simulink subsystem "simscape_thermofluids_full_subsystem"  (R2024b)
settings: Solver=VariableStepAuto  StartTime=0.0  StopTime=10.0  RelTol=1e-3
values from neighbouring files (symbols this model uses):
  Ambient_temp = 300    [design_details.m]
  hose_length = 20    [design_details.m]
  Initial_temp = 300    [design_details.m]
  mass_per_length_return = steel_density*wall_thickness*(return_pipe_inner_area + return_pipe_outer_area)    [design_details.m]
  mass_per_length_supply = steel_density*wall_thickness*(supply_pipe_inner_area + supply_pipe_outer_area)    [design_details.m]
  return_pipe_inner_diameter = 0.1    [design_details.m]
  supply_pipe_inner_diameter = 0.1    [design_details.m]
  wall_thickness = 2/1000    (= 0.002)    [design_details.m]
undefined symbols (not defined in the file or in its folder): AC_bypass_line_Mdot, AC_bypass_line_Qdot, AC_Bypass_SOV_POS, AC_Engine_SOV_POS, AC_return_coupling_Qdot, AC_return_line_Mdot, AC_return_line_Qdot, AC_Return_SOV_POS, AC_supply_coupling_Qdot, AC_supply_line_Mdot, AC_supply_line_Qdot, AC_Supply_SOV_POS, AC_Tank_return_line_mdot, AC_Tank_return_line_Qdot, AC_TANK_SUPPLY_LINE_MDOT, AC_TANK_SUPPLY_LINE_QDOT, AC_Tank_Vent_mdot, AC_Tank_Vent_Qdot, Engine_feed_mdot, Engine_feed_Qdot, GH2_PROP_VALVE_POS, GS_GH2_RETURN_PROP_POS, GS_GH2_RETURN_SOV_POS, GS_GH2_SOV_POS, GS_LH2_Return_SOV_POS, GS_RETURN_PROP_POS, GS_Supply_SOV_POS, LH2_PROP_VALVE_POS, P_BYPASS, P_COUPLING_AC, P_COUPLING_AC_RETURN, P_COUPLINGS_GS, P_ENGINE_FEED, P_GAS_RETURN, P_GH2_SUPPLY_GS, P_HOSE_GS, P_HOSE_RETURN_GS, P_PUMP_GS, P_TANK_AC, P_TANK_GS, P_VALVE_GS, P_VALVE_RETURN_GS, T_BYPASS, T_COUPLING_AC, T_COUPLING_AC_RETURN, T_COUPLINGS_GS, T_ENGINE_FEED, T_GAS_RETURN, T_GH2_SUPPLY_GS, T_HOSE_GS, T_HOSE_RETURN_GS, T_PUMP_GS, T_TANK_AC, T_TANK_GS, T_VALVE_GS, T_VALVE_RETURN_GS
libraries: nesl_utility x85, fl_lib x83, SimscapeFluids_lib x17
(part 1 of 2)
settings Model: Creator=MW  LastModifiedBy=MW

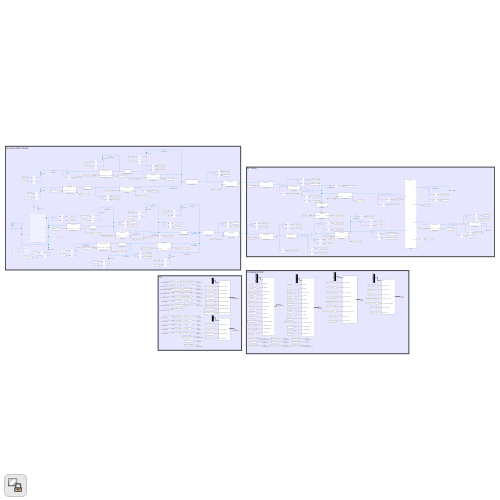
[thumbnail: Simulink's stored preview of the top-level diagram]
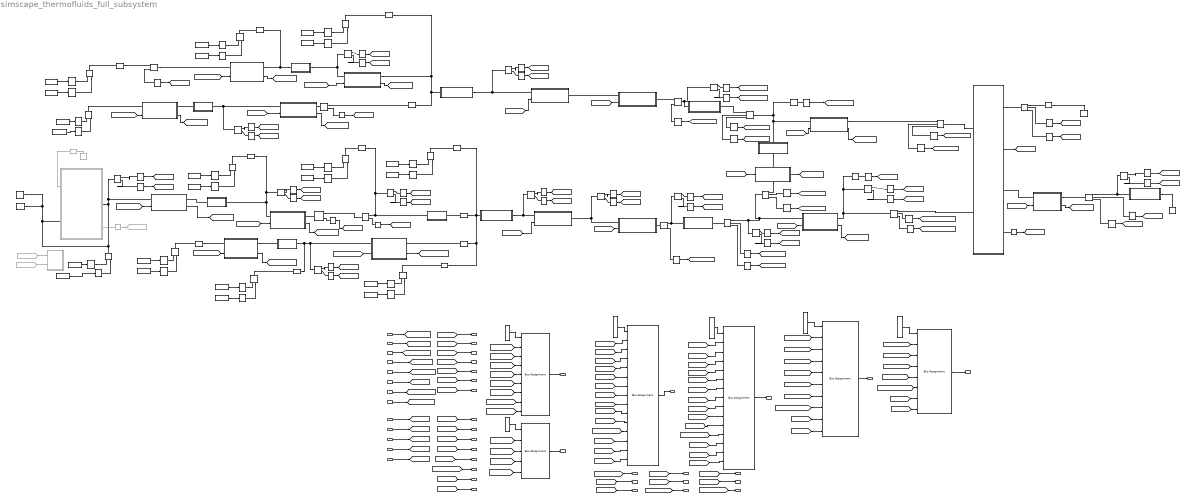
== system simscape_thermofluids_full_subsystem ==
  note: AC fluids
  note: Ground station fluids
  note: DIAGNOSTICS
  note: I/O
  LH2_PROP_VALVE_CMD : Inport  OutDataTypeStr=double
  GH2_PROP_VALVE_CMD : Inport  Port=2
  LH2 VENT PROP VALVE CMD : Inport  Port=3
  GS_LH2_Supply_SOV_CMD : Inport  Port=4  OutDataTypeStr=boolean
  GS_LH2_Return_SOV_CMD : Inport  Port=5  OutDataTypeStr=boolean
  GS_GH2_SOV_CMD : Inport  Port=6  OutDataTypeStr=boolean
  Couplings_connected : Inport  Port=7  OutDataTypeStr=boolean
  AC_Bypass_SOV_CMD : Inport  Port=8  OutDataTypeStr=boolean
  AC_Supply_SOV_CMD : Inport  Port=9  OutDataTypeStr=boolean
  AC_Return_SOV_CMD : Inport  Port=10  OutDataTypeStr=boolean
  AC_Engine_SOV_CMD : Inport  Port=11  OutDataTypeStr=boolean
  GS_GH2_RETURN_SOV_CMD : Inport  Port=12  OutDataTypeStr=boolean
  GH2_VENT_PROP_VALVE_CMD : Inport  Port=13
  AC bypass pipe : Subsystem  ReferencedSubsystem=AC_bypass_pipe
      settings: PortSchema="{\"entries\":[{\"content\":{\"sides\":[{\"content\":{},\"type\":\"ConnectorPlacement.EquallySpacedRectSide\",\"uuid\":\"f855fa5c-e5c1-49a4-a4bd-bb526208fa5d\"},{\"content\":{\"side\":\"RIGHT\"},\"type\":\"ConnectorPlacement.EquallySpacedRectSide\",\"uuid\":\"38379b5c-3270-47da-8350-930eb7311903\"},{\"content\":{\"connectorIds\":[\"RConn1\"],\"side\":\"TOP\"},\"type\":\"ConnectorPlacement.EquallySpacedRectSide\",\"uuid\":\"bb5b7562-7a02-4290-8016-95c457fb0f4b\"},{\"content\":{\"connectorIds\":[\"LConn1\"],\"side\":\"BOTTOM\"},\"type\":\"ConnectorPlacement.EquallySpacedRectSide\",\"uuid\":\"44fc2626-0acf-483b-8317-5c56b92a9255\"}]},\"type\":\"ConnectorPlacement.EquallySpacedConnector\",\"uuid\":\"6c85636f-b857-4cac-a183-27922e813604\"}],\"packageUris\":[\"http://schema.mathworks.com/mf0/Connector/R2020b\"],\"version\":\"1.0\"}"
  AC engine feed pipe : Subsystem  ReferencedSubsystem=AC_engine_line_pipe
  AC return line pipe : Subsystem  ReferencedSubsystem=AC_return_line_pipe
  AC return vapour quality : fl_lib/Two-Phase Fluid/Sensors/Vapor Quality Sensor (2P)  vapor_fraction_spec=foundation.enum.vapor_fraction_spec.quality
      settings: InternalSimscapePortConfiguration="{\"Bottom\":[],\"Left\":[{\"id\":\"A\",\"label\":\"A\",\"type\":\"foundation.two_phase_fluid.two_phase_fluid\"}],\"Right\":[{\"id\":\"X\",\"label\":\"X\",\"type\":\"output\"}],\"Top\":[]}"
  AC supply line quality : fl_lib/Two-Phase Fluid/Sensors/Vapor Quality Sensor (2P)  vapor_fraction_spec=foundation.enum.vapor_fraction_spec.quality
      settings: InternalSimscapePortConfiguration="{\"Bottom\":[],\"Left\":[{\"id\":\"A\",\"label\":\"A\",\"type\":\"foundation.two_phase_fluid.two_phase_fluid\"}],\"Right\":[{\"id\":\"X\",\"label\":\"X\",\"type\":\"output\"}],\"Top\":[]}"
  AC tank : Subsystem  ReferencedSubsystem=AC_tank
      settings: PortSchema="{\"entries\":[{\"content\":{\"sides\":[{\"content\":{\"connectorIds\":[\"LConn1\",\"LConn2\"]},\"type\":\"ConnectorPlacement.EquallySpacedRectSide\",\"uuid\":\"18fbfd65-7892-4f33-871e-6daf68ba144c\"},{\"content\":{\"connectorIds\":[\"RConn1\",\"Out1\",\"RConn2\",\"RConn3\"],\"side\":\"RIGHT\"},\"type\":\"ConnectorPlacement.EquallySpacedRectSide\",\"uuid\":\"09c519c2-126c-4ac0-b88b-b8c0f8bd496e\"},{\"content\":{\"side\":\"TOP\"},\"type\":\"ConnectorPlacement.EquallySpacedRectSide\",\"uuid\":\"0da44e65-d94a-4bbc-a863-04d0cc4fadcc\"}]},\"type\":\"ConnectorPlacement.EquallySpacedConnector\",\"uuid\":\"f3f4eab3-fa1f-4341-9602-c44ab5467c31\"}],\"packageUris\":[\"http://schema.mathworks.com/mf0/Connector/R2020b\"],\"version\":\"1.0\"}"
  AC tank safety valve : SimscapeFluids_lib/Two-Phase Fluid/Valves & Orifices/Directional Control Valves/Check Valve (2P)  liquid_valve_parameterization=fluids.two_phase_fluid.valves_orifices.enum.LiquidPressureValveParameterization.LinearArea  opening_pressure_spec=fluids.two_phase_fluid.valves_orifices.enum.PressureControlSpec.PressureDifferential  p_crack_differential=4.5 bar  p_crack_gauge=0.1 MPa  p_max_differential=4.9 bar  p_max_gauge=0.2 MPa  mdot_nominal_max=0.1 kg/s  delta_p_nominal_max=0.001 MPa  valve_area_max=AC_vent_valve_orifice_area m^2  p_diff_TLU=[0.2 : 0.2 : 1.2] MPa  p_gauge_TLU=[0.2 : 0.2 : 1.2] MPa  valve_area_TLU=[1e-10, 2e-06, 4e-06, 6e-06, 8e-06, 1e-05] m^2  energy_spec=foundation.enum.energy_spec.temperature  p_inlet=0.101325 MPa  T_inlet=293.15 K  x_inlet=0  alpha_inlet=0  h_inlet=400 kJ/kg  u_inlet=400 kJ/kg  Cd=AC_vent_valve_discharge_coeff  pressure_recovery=false  leakage_fraction=1e-9  smoothing_factor=0.01  B_lam=0.999  tau_x=0.1 s  area=AC_vent_line_port_inner_area m^2  vapor_valve_parameterization=fluids.two_phase_fluid.valves_orifices.enum.VaporOrificeParameterization.Cv  opening_characteristic=fluids.two_phase_fluid.valves_orifices.enum.OpeningCharacteristics.Linear  Cv_max=4  p_diff_Cv_TLU=0.2 : 0.2 : 1.2 MPa  p_gauge_Cv_TLU=0.2 : 0.2 : 1.2 MPa  Cv_TLU=[1e-06, .8, 1.6, 2.4, 3.2, 4]  xT_Cv=0.7  Kv_max=3.6  p_diff_Kv_TLU=0.2 : 0.2 : 1.2 MPa  p_gauge_Kv_TLU=0.2 : 0.2 : 1.2 MPa  Kv_TLU=[1e-06, .72, 1.44, 2.16, 2.88, 3.6]  xT_Kv=0.7  orifice_area_max=1e-4 m^2  p_diff_orifice_area_TLU=0.2 : 0.2 : 1.2 MPa  p_gauge_orifice_area_TLU=0.2 : 0.2 : 1.2 MPa  orifice_area_TLU=[1e-10, 2e-05, 4e-05, 6e-05, 8e-05, .0001] m^2
      settings: InternalSimscapePortConfiguration="{\"Bottom\":[],\"Left\":[{\"id\":\"A\",\"label\":\"A\",\"type\":\"foundation.two_phase_fluid.two_phase_fluid\"}],\"Right\":[{\"id\":\"B\",\"label\":\"B\",\"type\":\"foundation.two_phase_fluid.two_phase_fluid\"}],\"Top\":[]}"
  AC_Bypass_SOV : Subsystem  ReferencedSubsystem=AC_return_SOV
      settings: PortSchema="{\"entries\":[{\"content\":{\"sides\":[{\"content\":{\"connectorIds\":[\"In1\"]},\"type\":\"ConnectorPlacement.EquallySpacedRectSide\",\"uuid\":\"7761104f-7ea1-4b82-8256-1f0a81ecff04\"},{\"content\":{\"connectorIds\":[\"Out1\"],\"side\":\"RIGHT\"},\"type\":\"ConnectorPlacement.EquallySpacedRectSide\",\"uuid\":\"77ad54b1-fc7d-49b0-961f-dd624ba54eaa\"},{\"content\":{\"connectorIds\":[\"RConn1\"],\"side\":\"TOP\"},\"type\":\"ConnectorPlacement.EquallySpacedRectSide\",\"uuid\":\"3eb2c4da-9d99-4a14-9c12-4cb71cddfd05\"},{\"content\":{\"connectorIds\":[\"LConn1\"],\"side\":\"BOTTOM\"},\"type\":\"ConnectorPlacement.EquallySpacedRectSide\",\"uuid\":\"cc93d467-c3c5-4ce4-93ce-594b4fdbf767\"}]},\"type\":\"ConnectorPlacement.EquallySpacedConnector\",\"uuid\":\"a385487e-9e14-4b1e-bbba-76ef306222d1\"}],\"packageUris\":[\"http://schema.mathworks.com/mf0/Connector/R2020b\"],\"version\":\"1.0\"}"
  AC_Engine_SOV : Subsystem  ReferencedSubsystem=AC_Engine_SOV
      settings: PortSchema="{\"entries\":[{\"content\":{\"sides\":[{\"content\":{\"connectorIds\":[\"LConn1\",\"In1\"]},\"type\":\"ConnectorPlacement.EquallySpacedRectSide\",\"uuid\":\"8de00a24-9637-44f9-b77e-5b0008e83c26\"},{\"content\":{\"connectorIds\":[\"RConn1\",\"Out1\"],\"side\":\"RIGHT\"},\"type\":\"ConnectorPlacement.EquallySpacedRectSide\",\"uuid\":\"a538d446-b2a2-4ee6-8065-c38203dba177\"},{\"content\":{\"side\":\"TOP\"},\"type\":\"ConnectorPlacement.EquallySpacedRectSide\",\"uuid\":\"7c3a0b8e-131f-419e-9dd3-9151f58d9c4d\"}]},\"type\":\"ConnectorPlacement.EquallySpacedConnector\",\"uuid\":\"82546791-8f2d-494c-94b0-dfe79e322a77\"}],\"packageUris\":[\"http://schema.mathworks.com/mf0/Connector/R2020b\"],\"version\":\"1.0\"}"
  AC_Return_Coupling : Subsystem  ReferencedSubsystem=Return_coupling
      settings: PortSchema="{\"entries\":[{\"content\":{\"sides\":[{\"content\":{\"connectorIds\":[\"LConn1\",\"In1\"]},\"type\":\"ConnectorPlacement.EquallySpacedRectSide\",\"uuid\":\"1377ff57-d661-4db4-88bf-068b5be5647d\"},{\"content\":{\"connectorIds\":[\"RConn1\"],\"side\":\"RIGHT\"},\"type\":\"ConnectorPlacement.EquallySpacedRectSide\",\"uuid\":\"b2bd98a1-a4a4-4b83-ae68-33d4546d1bd4\"},{\"content\":{\"side\":\"TOP\"},\"type\":\"ConnectorPlacement.EquallySpacedRectSide\",\"uuid\":\"bd2d13e7-0124-4459-acb6-2626b7f191a3\"}]},\"type\":\"ConnectorPlacement.EquallySpacedConnector\",\"uuid\":\"1a0dd594-d6c0-4a46-87d8-aae9dae4eba9\"}],\"packageUris\":[\"http://schema.mathworks.com/mf0/Connector/R2020b\"],\"version\":\"1.0\"}"
  AC_Return_SOV : Subsystem
      settings: PortSchema="{\"entries\":[{\"content\":{\"sides\":[{\"content\":{\"connectorIds\":[\"LConn1\",\"In1\"]},\"type\":\"ConnectorPlacement.EquallySpacedRectSide\",\"uuid\":\"1377ff57-d661-4db4-88bf-068b5be5647d\"},{\"content\":{\"connectorIds\":[\"RConn1\",\"Out1\"],\"side\":\"RIGHT\"},\"type\":\"ConnectorPlacement.EquallySpacedRectSide\",\"uuid\":\"b2bd98a1-a4a4-4b83-ae68-33d4546d1bd4\"},{\"content\":{\"side\":\"TOP\"},\"type\":\"ConnectorPlacement.EquallySpacedRectSide\",\"uuid\":\"bd2d13e7-0124-4459-acb6-2626b7f191a3\"},{\"content\":{\"side\":\"BOTTOM\"},\"type\":\"ConnectorPlacement.EquallySpacedRectSide\",\"uuid\":\"65261db1-7dc3-4c3c-a5c1-ee0ef291cfbc\"}]},\"type\":\"ConnectorPlacement.EquallySpacedConnector\",\"uuid\":\"1a0dd594-d6c0-4a46-87d8-aae9dae4eba9\"}],\"packageUris\":[\"http://schema.mathworks.com/mf0/Connector/R2020b\"],\"version\":\"1.0\"}"
  AC_Supply_Coupling : Subsystem  ReferencedSubsystem=Supply_coupling
      settings: PortSchema="{\"entries\":[{\"content\":{\"sides\":[{\"content\":{\"connectorIds\":[\"LConn1\",\"In1\"]},\"type\":\"ConnectorPlacement.EquallySpacedRectSide\",\"uuid\":\"1377ff57-d661-4db4-88bf-068b5be5647d\"},{\"content\":{\"connectorIds\":[\"RConn1\"],\"side\":\"RIGHT\"},\"type\":\"ConnectorPlacement.EquallySpacedRectSide\",\"uuid\":\"b2bd98a1-a4a4-4b83-ae68-33d4546d1bd4\"},{\"content\":{\"side\":\"TOP\"},\"type\":\"ConnectorPlacement.EquallySpacedRectSide\",\"uuid\":\"bd2d13e7-0124-4459-acb6-2626b7f191a3\"}]},\"type\":\"ConnectorPlacement.EquallySpacedConnector\",\"uuid\":\"1a0dd594-d6c0-4a46-87d8-aae9dae4eba9\"}],\"packageUris\":[\"http://schema.mathworks.com/mf0/Connector/R2020b\"],\"version\":\"1.0\"}"
  AC_Supply_SOV : Subsystem  ReferencedSubsystem=AC_supply_SOV
      settings: PortSchema="{\"entries\":[{\"content\":{\"sides\":[{\"content\":{\"connectorIds\":[\"LConn1\",\"In1\"]},\"type\":\"ConnectorPlacement.EquallySpacedRectSide\",\"uuid\":\"7761104f-7ea1-4b82-8256-1f0a81ecff04\"},{\"content\":{\"connectorIds\":[\"RConn1\",\"Out1\"],\"side\":\"RIGHT\"},\"type\":\"ConnectorPlacement.EquallySpacedRectSide\",\"uuid\":\"77ad54b1-fc7d-49b0-961f-dd624ba54eaa\"},{\"content\":{\"side\":\"TOP\"},\"type\":\"ConnectorPlacement.EquallySpacedRectSide\",\"uuid\":\"3eb2c4da-9d99-4a14-9c12-4cb71cddfd05\"}]},\"type\":\"ConnectorPlacement.EquallySpacedConnector\",\"uuid\":\"a385487e-9e14-4b1e-bbba-76ef306222d1\"}],\"packageUris\":[\"http://schema.mathworks.com/mf0/Connector/R2020b\"],\"version\":\"1.0\"}"
  AC_supply_line_pipe : Subsystem  ReferencedSubsystem=AC_supply_line_pipe
  Atmosphere : fl_lib/Two-Phase Fluid/Elements/Reservoir (2P)  Commented=on  pressure_spec=foundation.enum.ReservoirPressureSpec2P.Specified  reservoir_pressure=0.101325 MPa  reservoir_condensing_temperature=373.15 K  reservoir_evaporating_temperature=373.15 K  energy_spec=foundation.enum.ReservoirEnergySpec2P.Temperature  reservoir_temperature=Ambient_temp K  reservoir_quality=0.5  reservoir_void_fraction=0.5  reservoir_enthalpy=1500 kJ/kg  reservoir_internal_energy=1500 kJ/kg  reservoir_subcooling=5 deltaK  reservoir_superheating=5 deltaK  area_A=0.01 m^2
  Atmosphere2 : fl_lib/Two-Phase Fluid/Elements/Reservoir (2P)  pressure_spec=foundation.enum.ReservoirPressureSpec2P.Specified  reservoir_pressure=0.101325 MPa  reservoir_condensing_temperature=373.15 K  reservoir_evaporating_temperature=373.15 K  energy_spec=foundation.enum.ReservoirEnergySpec2P.Temperature  reservoir_temperature=293.15 K  reservoir_quality=0.5  reservoir_void_fraction=0.5  reservoir_enthalpy=1500 kJ/kg  reservoir_internal_energy=1500 kJ/kg  reservoir_subcooling=5 deltaK  reservoir_superheating=5 deltaK  area_A=0.02 m^2
  Bus Assignment : BusAssignment  AssignedSignals=P_TANK_GS,P_PUMP_GS,P_GH2_SUPPLY_GS,P_VALVE_GS,P_HOSE_GS,P_COUPLINGS_GS,P_COUPLING_AC,P_BYPASS,P_TANK_AC,P_ENGINE_FEED,P_COUPLING_AC_RETURN,P_HOSE_RETURN_GS,P_VALVE_RETURN_GS,P_GAS_RETURN
  Bus Assignment1 : BusAssignment  AssignedSignals=T_TANK_GS,T_PUMP_GS,T_GH2_SUPPLY_GS,T_VALVE_GS,T_HOSE_GS,T_COUPLINGS_GS,T_COUPLING_AC,T_BYPASS,T_TANK_AC,T_ENGINE_FEED,T_COUPLING_AC_RETURN,T_HOSE_RETURN_GS,T_VALVE_RETURN_GS,T_GAS_RETURN
  Bus Assignment2 : BusAssignment  AssignedSignals=LH2_PROP_VALVE_POS,GH2_PROP_VALVE_POS,GS_Supply_SOV_POS,GS_GH2_SOV_POS,GS_LH2_Return_SOV_POS,GS_RETURN_PROP_POS,GS_GH2_RETURN_PROP_POS,GS_GH2_RETURN_SOV_POS
  Bus Assignment3 : BusAssignment  AssignedSignals=AC_Return_SOV_POS,AC_Supply_SOV_POS,AC_Bypass_SOV_POS,AC_Engine_SOV_POS
  Bus Assignment4 : BusAssignment  AssignedSignals=AC_supply_line_Qdot,AC_return_line_Qdot,AC_return_coupling_Qdot,AC_supply_coupling_Qdot,AC_bypass_line_Qdot,AC_Tank_return_line_Qdot,AC_TANK_SUPPLY_LINE_QDOT,Engine_feed_Qdot,AC_Tank_Vent_Qdot
  Bus Assignment5 : BusAssignment  AssignedSignals=AC_supply_line_Mdot,AC_bypass_line_Mdot,AC_return_line_Mdot,AC_Tank_return_line_mdot,AC_TANK_SUPPLY_LINE_MDOT,AC_Tank_Vent_mdot,Engine_feed_mdot
  Bus Creator : BusCreator  Inputs=14  OutDataTypeStr=Bus: P_DIAGNOSTIC  NonVirtualBus=on
      settings: InheritFromInputs=off
  Bus Creator1 : BusCreator  Inputs=14  OutDataTypeStr=Bus: T_DIAGNOSTIC  NonVirtualBus=on
      settings: InheritFromInputs=off
  Bus Creator2 : BusCreator  Inputs=8  OutDataTypeStr=Bus: GS_VALVE_FEEDBACK  NonVirtualBus=on
      settings: InheritFromInputs=off
  Bus Creator3 : BusCreator  Inputs=4  OutDataTypeStr=Bus: AC_VALVE_FEEDBACK  NonVirtualBus=on
      settings: InheritFromInputs=off
  Bus Creator4 : BusCreator  Inputs=9  OutDataTypeStr=Bus: AC_QDOT  NonVirtualBus=on
      settings: InheritFromInputs=off
  Bus Creator5 : BusCreator  Inputs=7  OutDataTypeStr=Bus: AC_MDOT  NonVirtualBus=on
      settings: InheritFromInputs=off
  Constant1 : Constant  Value=20
  Constant10 : Constant  Value=0.15
  Constant{2..3,8,11,13,15,17,19,21} (9 alike) : Constant  Value=Ambient_temp
  Constant{5,7,12,14,16,18,20,22} (8 alike) : Constant  Value=0.1013
  Constant4 : Constant  Value=0.5
  Constant6 : Constant  Value=20
  Constant9 : Constant  Value=0.5
  Flow Rate Sensor (2P){1..6,8..10} (9 alike) : fl_lib/Two-Phase Fluid/Sensors/Flow Rate Sensor (2P)  mass_flow_measure=true  volumetric_flow_measure=true  energy_flow_measure=false
      settings: InternalSimscapePortConfiguration="{\"Bottom\":[],\"Left\":[{\"id\":\"A\",\"label\":\"A\",\"type\":\"foundation.two_phase_fluid.two_phase_fluid\"}],\"Right\":[{\"id\":\"B\",\"label\":\"B\",\"type\":\"foundation.two_phase_fluid.two_phase_fluid\"},{\"id\":\"M\",\"label\":\"M\",\"type\":\"output\"},{\"id\":\"V\",\"label\":\"V\",\"type\":\"output\"}],\"Top\":[]}"
  Flow Rate Sensor (2P)7 : fl_lib/Two-Phase Fluid/Sensors/Flow Rate Sensor (2P)  mass_flow_measure=false  volumetric_flow_measure=true  energy_flow_measure=false
      settings: InternalSimscapePortConfiguration="{\"Bottom\":[],\"Left\":[{\"id\":\"A\",\"label\":\"A\",\"type\":\"foundation.two_phase_fluid.two_phase_fluid\"}],\"Right\":[{\"id\":\"B\",\"label\":\"B\",\"type\":\"foundation.two_phase_fluid.two_phase_fluid\"},{\"id\":\"V\",\"label\":\"V\",\"type\":\"output\"}],\"Top\":[]}"
  Flow rate sensor : fl_lib/Two-Phase Fluid/Sensors/Flow Rate Sensor (2P)  mass_flow_measure=true  volumetric_flow_measure=false  energy_flow_measure=false
      settings: InternalSimscapePortConfiguration="{\"Bottom\":[],\"Left\":[{\"id\":\"A\",\"label\":\"A\",\"type\":\"foundation.two_phase_fluid.two_phase_fluid\"}],\"Right\":[{\"id\":\"B\",\"label\":\"B\",\"type\":\"foundation.two_phase_fluid.two_phase_fluid\"},{\"id\":\"M\",\"label\":\"M\",\"type\":\"output\"}],\"Top\":[]}"
  From : From  Commented=on  GotoTag=Target_tank_pressure
  From14 : From  Commented=on  GotoTag=GS_tank_pressure
  GH2 Proportional valve : Subsystem  ReferencedSubsystem=Gas_prop_valve
      settings: PortSchema="{\"entries\":[{\"content\":{\"sides\":[{\"content\":{\"connectorIds\":[\"LConn1\",\"In1\"]},\"type\":\"ConnectorPlacement.EquallySpacedRectSide\",\"uuid\":\"7761104f-7ea1-4b82-8256-1f0a81ecff04\"},{\"content\":{\"connectorIds\":[\"LConn2\",\"Out1\"],\"side\":\"RIGHT\"},\"type\":\"ConnectorPlacement.EquallySpacedRectSide\",\"uuid\":\"77ad54b1-fc7d-49b0-961f-dd624ba54eaa\"},{\"content\":{\"side\":\"TOP\"},\"type\":\"ConnectorPlacement.EquallySpacedRectSide\",\"uuid\":\"3eb2c4da-9d99-4a14-9c12-4cb71cddfd05\"},{\"content\":{\"side\":\"BOTTOM\"},\"type\":\"ConnectorPlacement.EquallySpacedRectSide\",\"uuid\":\"e49cc93b-8c4a-4262-8b13-a5abe2820965\"}]},\"type\":\"ConnectorPlacement.EquallySpacedConnector\",\"uuid\":\"a385487e-9e14-4b1e-bbba-76ef306222d1\"}],\"packageUris\":[\"http://schema.mathworks.com/mf0/Connector/R2020b\"],\"version\":\"1.0\"}"
  GH2 return check valve : SimscapeFluids_lib/Two-Phase Fluid/Valves & Orifices/Directional Control Valves/Check Valve (2P)  liquid_valve_parameterization=fluids.two_phase_fluid.valves_orifices.enum.LiquidPressureValveParameterization.LinearArea  opening_pressure_spec=fluids.two_phase_fluid.valves_orifices.enum.PressureControlSpec.PressureDifferential  p_crack_differential=0.01 bar  p_crack_gauge=0.1 MPa  p_max_differential=0.03 bar  p_max_gauge=0.2 MPa  mdot_nominal_max=0.1 kg/s  delta_p_nominal_max=0.001 MPa  valve_area_max=supply_valve_orifice_area m^2  p_diff_TLU=[0.2 : 0.2 : 1.2] MPa  p_gauge_TLU=[0.2 : 0.2 : 1.2] MPa  valve_area_TLU=[1e-10, 2e-06, 4e-06, 6e-06, 8e-06, 1e-05] m^2  energy_spec=foundation.enum.energy_spec.temperature  p_inlet=0.101325 MPa  T_inlet=293.15 K  x_inlet=0  alpha_inlet=0  h_inlet=400 kJ/kg  u_inlet=400 kJ/kg  Cd=0.8  pressure_recovery=false  leakage_fraction=1e-9  smoothing_factor=0.01  B_lam=valve_laminar_p_ratio  tau_x=0.1 s  area=supply_pipe_inner_area m^2  vapor_valve_parameterization=fluids.two_phase_fluid.valves_orifices.enum.VaporOrificeParameterization.Cv  opening_characteristic=fluids.two_phase_fluid.valves_orifices.enum.OpeningCharacteristics.Linear  Cv_max=4  p_diff_Cv_TLU=0.2 : 0.2 : 1.2 MPa  p_gauge_Cv_TLU=0.2 : 0.2 : 1.2 MPa  Cv_TLU=[1e-06, .8, 1.6, 2.4, 3.2, 4]  xT_Cv=0.7  Kv_max=3.6  p_diff_Kv_TLU=0.2 : 0.2 : 1.2 MPa  p_gauge_Kv_TLU=0.2 : 0.2 : 1.2 MPa  Kv_TLU=[1e-06, .72, 1.44, 2.16, 2.88, 3.6]  xT_Kv=0.7  orifice_area_max=1e-4 m^2  p_diff_orifice_area_TLU=0.2 : 0.2 : 1.2 MPa  p_gauge_orifice_area_TLU=0.2 : 0.2 : 1.2 MPa  orifice_area_TLU=[1e-10, 2e-05, 4e-05, 6e-05, 8e-05, .0001] m^2
      settings: InternalSimscapePortConfiguration="{\"Bottom\":[],\"Left\":[{\"id\":\"A\",\"label\":\"A\",\"type\":\"foundation.two_phase_fluid.two_phase_fluid\"}],\"Right\":[{\"id\":\"B\",\"label\":\"B\",\"type\":\"foundation.two_phase_fluid.two_phase_fluid\"}],\"Top\":[]}"
  GH2 return check valve1 : SimscapeFluids_lib/Two-Phase Fluid/Valves & Orifices/Directional Control Valves/Check Valve (2P)  liquid_valve_parameterization=fluids.two_phase_fluid.valves_orifices.enum.LiquidPressureValveParameterization.LinearArea  opening_pressure_spec=fluids.two_phase_fluid.valves_orifices.enum.PressureControlSpec.PressureDifferential  p_crack_differential=0.01 bar  p_crack_gauge=0.1 MPa  p_max_differential=0.03 bar  p_max_gauge=0.2 MPa  mdot_nominal_max=0.1 kg/s  delta_p_nominal_max=0.001 MPa  valve_area_max=supply_valve_orifice_area m^2  p_diff_TLU=[0.2 : 0.2 : 1.2] MPa  p_gauge_TLU=[0.2 : 0.2 : 1.2] MPa  valve_area_TLU=[1e-10, 2e-06, 4e-06, 6e-06, 8e-06, 1e-05] m^2  energy_spec=foundation.enum.energy_spec.temperature  p_inlet=0.101325 MPa  T_inlet=293.15 K  x_inlet=0  alpha_inlet=0  h_inlet=400 kJ/kg  u_inlet=400 kJ/kg  Cd=0.8  pressure_recovery=false  leakage_fraction=1e-9  smoothing_factor=0.01  B_lam=valve_laminar_p_ratio  tau_x=0.1 s  area=supply_pipe_inner_area m^2  vapor_valve_parameterization=fluids.two_phase_fluid.valves_orifices.enum.VaporOrificeParameterization.Cv  opening_characteristic=fluids.two_phase_fluid.valves_orifices.enum.OpeningCharacteristics.Linear  Cv_max=4  p_diff_Cv_TLU=0.2 : 0.2 : 1.2 MPa  p_gauge_Cv_TLU=0.2 : 0.2 : 1.2 MPa  Cv_TLU=[1e-06, .8, 1.6, 2.4, 3.2, 4]  xT_Cv=0.7  Kv_max=3.6  p_diff_Kv_TLU=0.2 : 0.2 : 1.2 MPa  p_gauge_Kv_TLU=0.2 : 0.2 : 1.2 MPa  Kv_TLU=[1e-06, .72, 1.44, 2.16, 2.88, 3.6]  xT_Kv=0.7  orifice_area_max=1e-4 m^2  p_diff_orifice_area_TLU=0.2 : 0.2 : 1.2 MPa  p_gauge_orifice_area_TLU=0.2 : 0.2 : 1.2 MPa  orifice_area_TLU=[1e-10, 2e-05, 4e-05, 6e-05, 8e-05, .0001] m^2
      settings: InternalSimscapePortConfiguration="{\"Bottom\":[],\"Left\":[{\"id\":\"A\",\"label\":\"A\",\"type\":\"foundation.two_phase_fluid.two_phase_fluid\"}],\"Right\":[{\"id\":\"B\",\"label\":\"B\",\"type\":\"foundation.two_phase_fluid.two_phase_fluid\"}],\"Top\":[]}"
  GH2 source1 : fl_lib/Two-Phase Fluid/Elements/Controlled Reservoir (2P)  pressure_spec=foundation.enum.ControlledReservoirPressureSpec2P.Specified  energy_spec=foundation.enum.ControlledReservoirEnergySpec2P.VaporTemperature  area_A=supply_valve_orifice_area m^2  pressure_limit_spec=foundation.enum.PressureLimitSpec2P.Warn
      settings: InternalSimscapePortConfiguration="{\"Bottom\":[],\"Left\":[{\"id\":\"A\",\"label\":\"A\",\"type\":\"foundation.two_phase_fluid.two_phase_fluid\"}],\"Right\":[{\"id\":\"T\",\"label\":\"T\",\"type\":\"input\"},{\"id\":\"P\",\"label\":\"P\",\"type\":\"input\"}],\"Top\":[]}"
  GH2 supply check valve : SimscapeFluids_lib/Two-Phase Fluid/Valves & Orifices/Directional Control Valves/Check Valve (2P)  liquid_valve_parameterization=fluids.two_phase_fluid.valves_orifices.enum.LiquidPressureValveParameterization.LinearArea  opening_pressure_spec=fluids.two_phase_fluid.valves_orifices.enum.PressureControlSpec.PressureDifferential  p_crack_differential=0.01 bar  p_crack_gauge=0.1 MPa  p_max_differential=0.03 bar  p_max_gauge=0.2 MPa  mdot_nominal_max=0.1 kg/s  delta_p_nominal_max=0.001 MPa  valve_area_max=supply_valve_orifice_area m^2  p_diff_TLU=[0.2 : 0.2 : 1.2] MPa  p_gauge_TLU=[0.2 : 0.2 : 1.2] MPa  valve_area_TLU=[1e-10, 2e-06, 4e-06, 6e-06, 8e-06, 1e-05] m^2  energy_spec=foundation.enum.energy_spec.temperature  p_inlet=0.101325 MPa  T_inlet=293.15 K  x_inlet=0  alpha_inlet=0  h_inlet=400 kJ/kg  u_inlet=400 kJ/kg  Cd=0.8  pressure_recovery=false  leakage_fraction=1e-9  smoothing_factor=0.01  B_lam=valve_laminar_p_ratio  tau_x=0.1 s  area=supply_pipe_inner_area m^2  vapor_valve_parameterization=fluids.two_phase_fluid.valves_orifices.enum.VaporOrificeParameterization.Cv  opening_characteristic=fluids.two_phase_fluid.valves_orifices.enum.OpeningCharacteristics.Linear  Cv_max=4  p_diff_Cv_TLU=0.2 : 0.2 : 1.2 MPa  p_gauge_Cv_TLU=0.2 : 0.2 : 1.2 MPa  Cv_TLU=[1e-06, .8, 1.6, 2.4, 3.2, 4]  xT_Cv=0.7  Kv_max=3.6  p_diff_Kv_TLU=0.2 : 0.2 : 1.2 MPa  p_gauge_Kv_TLU=0.2 : 0.2 : 1.2 MPa  Kv_TLU=[1e-06, .72, 1.44, 2.16, 2.88, 3.6]  xT_Kv=0.7  orifice_area_max=1e-4 m^2  p_diff_orifice_area_TLU=0.2 : 0.2 : 1.2 MPa  p_gauge_orifice_area_TLU=0.2 : 0.2 : 1.2 MPa  orifice_area_TLU=[1e-10, 2e-05, 4e-05, 6e-05, 8e-05, .0001] m^2
      settings: InternalSimscapePortConfiguration="{\"Bottom\":[],\"Left\":[{\"id\":\"A\",\"label\":\"A\",\"type\":\"foundation.two_phase_fluid.two_phase_fluid\"}],\"Right\":[{\"id\":\"B\",\"label\":\"B\",\"type\":\"foundation.two_phase_fluid.two_phase_fluid\"}],\"Top\":[]}"
  GH2 vent : fl_lib/Two-Phase Fluid/Elements/Controlled Reservoir (2P)  pressure_spec=foundation.enum.ControlledReservoirPressureSpec2P.Specified  energy_spec=foundation.enum.ControlledReservoirEnergySpec2P.VaporTemperature  area_A=supply_valve_orifice_area m^2  pressure_limit_spec=foundation.enum.PressureLimitSpec2P.Warn
      settings: InternalSimscapePortConfiguration="{\"Bottom\":[],\"Left\":[{\"id\":\"A\",\"label\":\"A\",\"type\":\"foundation.two_phase_fluid.two_phase_fluid\"}],\"Right\":[{\"id\":\"T\",\"label\":\"T\",\"type\":\"input\"},{\"id\":\"P\",\"label\":\"P\",\"type\":\"input\"}],\"Top\":[]}"
  GH2 vent proportional valve : Subsystem  ReferencedSubsystem=Return_gas_prop_valve
      settings: PortSchema="{\"entries\":[{\"content\":{\"sides\":[{\"content\":{\"connectorIds\":[\"LConn2\",\"In1\"]},\"type\":\"ConnectorPlacement.EquallySpacedRectSide\",\"uuid\":\"7b60590b-4a7b-465d-b616-9ce36d4c9bd1\"},{\"content\":{\"connectorIds\":[\"LConn1\",\"Out1\"],\"side\":\"RIGHT\"},\"type\":\"ConnectorPlacement.EquallySpacedRectSide\",\"uuid\":\"021f4d26-2a2b-40fc-b211-2c38ffe0620d\"},{\"content\":{\"side\":\"TOP\"},\"type\":\"ConnectorPlacement.EquallySpacedRectSide\",\"uuid\":\"273f71b8-2e8c-4f2f-b50f-0419d15b1792\"}]},\"type\":\"ConnectorPlacement.EquallySpacedConnector\",\"uuid\":\"b42a82ba-0baa-43b5-8ff8-ec1372f42070\"}],\"packageUris\":[\"http://schema.mathworks.com/mf0/Connector/R2020b\"],\"version\":\"1.0\"}"
  GH2 vent{1..7} (7 alike) : fl_lib/Two-Phase Fluid/Elements/Controlled Reservoir (2P)  pressure_spec=foundation.enum.ControlledReservoirPressureSpec2P.Specified  energy_spec=foundation.enum.ControlledReservoirEnergySpec2P.VaporTemperature  area_A=GS_vent_inner_area m^2  pressure_limit_spec=foundation.enum.PressureLimitSpec2P.Warn
      settings: InternalSimscapePortConfiguration="{\"Bottom\":[],\"Left\":[{\"id\":\"A\",\"label\":\"A\",\"type\":\"foundation.two_phase_fluid.two_phase_fluid\"}],\"Right\":[{\"id\":\"T\",\"label\":\"T\",\"type\":\"input\"},{\"id\":\"P\",\"label\":\"P\",\"type\":\"input\"}],\"Top\":[]}"
  GS GH2 SOV : Subsystem  ReferencedSubsystem=GS_return_SOV
      settings: PortSchema="{\"entries\":[{\"content\":{\"sides\":[{\"content\":{\"connectorIds\":[\"LConn1\",\"In1\"]},\"type\":\"ConnectorPlacement.EquallySpacedRectSide\",\"uuid\":\"60551d44-a89b-431d-905b-6466ad26fb96\"},{\"content\":{\"connectorIds\":[\"RConn1\",\"Out1\"],\"side\":\"RIGHT\"},\"type\":\"ConnectorPlacement.EquallySpacedRectSide\",\"uuid\":\"980db565-415c-49ff-806f-4e7ea1d33100\"},{\"content\":{\"side\":\"TOP\"},\"type\":\"ConnectorPlacement.EquallySpacedRectSide\",\"uuid\":\"073fdd51-397c-42b4-9e18-70e2190f3651\"}]},\"type\":\"ConnectorPlacement.EquallySpacedConnector\",\"uuid\":\"d12e0c08-f60f-4f0a-b617-0b9a29f01fdd\"}],\"packageUris\":[\"http://schema.mathworks.com/mf0/Connector/R2020b\"],\"version\":\"1.0\"}"
  GS LH2 Return SOV : Subsystem  ReferencedSubsystem=GS_return_SOV
      settings: PortSchema="{\"entries\":[{\"content\":{\"sides\":[{\"content\":{\"connectorIds\":[\"LConn1\",\"In1\"]},\"type\":\"ConnectorPlacement.EquallySpacedRectSide\",\"uuid\":\"60551d44-a89b-431d-905b-6466ad26fb96\"},{\"content\":{\"connectorIds\":[\"RConn1\",\"Out1\"],\"side\":\"RIGHT\"},\"type\":\"ConnectorPlacement.EquallySpacedRectSide\",\"uuid\":\"980db565-415c-49ff-806f-4e7ea1d33100\"},{\"content\":{\"side\":\"TOP\"},\"type\":\"ConnectorPlacement.EquallySpacedRectSide\",\"uuid\":\"073fdd51-397c-42b4-9e18-70e2190f3651\"}]},\"type\":\"ConnectorPlacement.EquallySpacedConnector\",\"uuid\":\"d12e0c08-f60f-4f0a-b617-0b9a29f01fdd\"}],\"packageUris\":[\"http://schema.mathworks.com/mf0/Connector/R2020b\"],\"version\":\"1.0\"}"
  GS return line pipe short : Subsystem
  GS return line pipe short2 : Subsystem
  GS supply line pipe : Subsystem
  GS supply line pipe short1 : Subsystem
  GS supply line pipe1 : Subsystem
  GS tank pressure controller : Subsystem  Commented=on
  GS_GH2_Return : Subsystem  ReferencedSubsystem=GS_supply_SOV
      settings: PortSchema="{\"entries\":[{\"content\":{\"sides\":[{\"content\":{\"connectorIds\":[\"LConn1\",\"In1\"]},\"type\":\"ConnectorPlacement.EquallySpacedRectSide\",\"uuid\":\"7761104f-7ea1-4b82-8256-1f0a81ecff04\"},{\"content\":{\"connectorIds\":[\"RConn1\",\"Out1\"],\"side\":\"RIGHT\"},\"type\":\"ConnectorPlacement.EquallySpacedRectSide\",\"uuid\":\"77ad54b1-fc7d-49b0-961f-dd624ba54eaa\"},{\"content\":{\"side\":\"TOP\"},\"type\":\"ConnectorPlacement.EquallySpacedRectSide\",\"uuid\":\"3eb2c4da-9d99-4a14-9c12-4cb71cddfd05\"}]},\"type\":\"ConnectorPlacement.EquallySpacedConnector\",\"uuid\":\"a385487e-9e14-4b1e-bbba-76ef306222d1\"}],\"packageUris\":[\"http://schema.mathworks.com/mf0/Connector/R2020b\"],\"version\":\"1.0\"}"
  GS_Return_Coupling : Subsystem  ReferencedSubsystem=Return_coupling
      settings: PortSchema="{\"entries\":[{\"content\":{\"sides\":[{\"content\":{\"connectorIds\":[\"LConn1\",\"In1\"]},\"type\":\"ConnectorPlacement.EquallySpacedRectSide\",\"uuid\":\"1377ff57-d661-4db4-88bf-068b5be5647d\"},{\"content\":{\"connectorIds\":[\"RConn1\"],\"side\":\"RIGHT\"},\"type\":\"ConnectorPlacement.EquallySpacedRectSide\",\"uuid\":\"b2bd98a1-a4a4-4b83-ae68-33d4546d1bd4\"},{\"content\":{\"side\":\"TOP\"},\"type\":\"ConnectorPlacement.EquallySpacedRectSide\",\"uuid\":\"bd2d13e7-0124-4459-acb6-2626b7f191a3\"}]},\"type\":\"ConnectorPlacement.EquallySpacedConnector\",\"uuid\":\"1a0dd594-d6c0-4a46-87d8-aae9dae4eba9\"}],\"packageUris\":[\"http://schema.mathworks.com/mf0/Connector/R2020b\"],\"version\":\"1.0\"}"
  GS_Supply_Coupling : Subsystem  ReferencedSubsystem=Supply_coupling
      settings: PortSchema="{\"entries\":[{\"content\":{\"sides\":[{\"content\":{\"connectorIds\":[\"LConn1\",\"In1\"]},\"type\":\"ConnectorPlacement.EquallySpacedRectSide\",\"uuid\":\"1377ff57-d661-4db4-88bf-068b5be5647d\"},{\"content\":{\"connectorIds\":[\"RConn1\"],\"side\":\"RIGHT\"},\"type\":\"ConnectorPlacement.EquallySpacedRectSide\",\"uuid\":\"b2bd98a1-a4a4-4b83-ae68-33d4546d1bd4\"},{\"content\":{\"side\":\"TOP\"},\"type\":\"ConnectorPlacement.EquallySpacedRectSide\",\"uuid\":\"bd2d13e7-0124-4459-acb6-2626b7f191a3\"}]},\"type\":\"ConnectorPlacement.EquallySpacedConnector\",\"uuid\":\"1a0dd594-d6c0-4a46-87d8-aae9dae4eba9\"}],\"packageUris\":[\"http://schema.mathworks.com/mf0/Connector/R2020b\"],\"version\":\"1.0\"}"
  GS_Supply_SOV : Subsystem  ReferencedSubsystem=GS_supply_SOV
      settings: PortSchema="{\"entries\":[{\"content\":{\"sides\":[{\"content\":{\"connectorIds\":[\"LConn1\",\"In1\"]},\"type\":\"ConnectorPlacement.EquallySpacedRectSide\",\"uuid\":\"7761104f-7ea1-4b82-8256-1f0a81ecff04\"},{\"content\":{\"connectorIds\":[\"RConn1\",\"Out1\"],\"side\":\"RIGHT\"},\"type\":\"ConnectorPlacement.EquallySpacedRectSide\",\"uuid\":\"77ad54b1-fc7d-49b0-961f-dd624ba54eaa\"},{\"content\":{\"side\":\"TOP\"},\"type\":\"ConnectorPlacement.EquallySpacedRectSide\",\"uuid\":\"3eb2c4da-9d99-4a14-9c12-4cb71cddfd05\"}]},\"type\":\"ConnectorPlacement.EquallySpacedConnector\",\"uuid\":\"a385487e-9e14-4b1e-bbba-76ef306222d1\"}],\"packageUris\":[\"http://schema.mathworks.com/mf0/Connector/R2020b\"],\"version\":\"1.0\"}"
  Goto1 : Goto  Commented=on  GotoTag=GROUND_GAUGE
  Ground station tank : Subsystem  Commented=on
  H2 2 phase : fl_lib/Two-Phase Fluid/Utilities/Two-Phase Fluid Properties (2P)  u_min=H2Tables.u_min kJ/kg  u_max=H2Tables.u_max kJ/kg  p_TLU=H2Tables.p MPa  p_crit=H2Tables.p_crit MPa  critical_region=foundation.enum.critical_region.clip  p_crit_fraction=0.12  p_atm=0.101325 MPa  properties_range_check=simscape.enum.assert.action.error  q_rev=0.01 Pa  unorm_liq=H2Tables.liquid.unorm  v_liq=H2Tables.liquid.v m^3/kg  s_liq=H2Tables.liquid.s kJ/(kg*K)  T_liq=H2Tables.liquid.T K  nu_liq=H2Tables.liquid.nu mm^2/s  k_liq=H2Tables.liquid.k W/(m*K)  Pr_liq=H2Tables.liquid.Pr  u_sat_liq=H2Tables.liquid.u_sat kJ/kg  unorm_vap=H2Tables.vapor.unorm  v_vap=H2Tables.vapor.v m^3/kg  s_vap=H2Tables.vapor.s kJ/(kg*K)  T_vap=H2Tables.vapor.T K  nu_vap=H2Tables.vapor.nu mm^2/s  k_vap=H2Tables.vapor.k W/(m*K)  Pr_vap=H2Tables.vapor.Pr  u_sat_vap=H2Tables.vapor.u_sat kJ/kg
      settings: InternalSimscapePortConfiguration="{\"Bottom\":[],\"Left\":[],\"Right\":[{\"id\":\"A\",\"label\":\"\",\"type\":\"foundation.two_phase_fluid.two_phase_fluid\"}],\"Top\":[]}"
  LH2 Proportional valve : Subsystem  ReferencedSubsystem=LH2_prop_valve
      settings: PortSchema="{\"entries\":[{\"content\":{\"sides\":[{\"content\":{\"connectorIds\":[\"LConn1\",\"In1\"]},\"type\":\"ConnectorPlacement.EquallySpacedRectSide\",\"uuid\":\"feebead4-63a3-41be-b6af-c9093fc48b74\"},{\"content\":{\"connectorIds\":[\"LConn2\",\"Out1\"],\"side\":\"RIGHT\"},\"type\":\"ConnectorPlacement.EquallySpacedRectSide\",\"uuid\":\"7fa0aa45-6202-479f-80c3-49b7dbf56766\"},{\"content\":{\"side\":\"TOP\"},\"type\":\"ConnectorPlacement.EquallySpacedRectSide\",\"uuid\":\"fffd3c2c-2b50-47ce-80c6-79193e21f29e\"},{\"content\":{\"side\":\"BOTTOM\"},\"type\":\"ConnectorPlacement.EquallySpacedRectSide\",\"uuid\":\"957ddecd-60b1-4a90-a8a1-75fcc228f543\"}]},\"type\":\"ConnectorPlacement.EquallySpacedConnector\",\"uuid\":\"476b1e20-77c8-4bf2-b4c4-536305065543\"}],\"packageUris\":[\"http://schema.mathworks.com/mf0/Connector/R2020b\"],\"version\":\"1.0\"}"
  LH2 recycle : fl_lib/Two-Phase Fluid/Elements/Controlled Reservoir (2P)  pressure_spec=foundation.enum.ControlledReservoirPressureSpec2P.Specified  energy_spec=foundation.enum.ControlledReservoirEnergySpec2P.LiquidTemperature  area_A=supply_valve_orifice_area m^2  pressure_limit_spec=foundation.enum.PressureLimitSpec2P.Warn
      settings: InternalSimscapePortConfiguration="{\"Bottom\":[],\"Left\":[{\"id\":\"A\",\"label\":\"A\",\"type\":\"foundation.two_phase_fluid.two_phase_fluid\"}],\"Right\":[{\"id\":\"T\",\"label\":\"T\",\"type\":\"input\"},{\"id\":\"P\",\"label\":\"P\",\"type\":\"input\"}],\"Top\":[]}"
  LH2 source : fl_lib/Two-Phase Fluid/Elements/Controlled Reservoir (2P)  pressure_spec=foundation.enum.ControlledReservoirPressureSpec2P.Specified  energy_spec=foundation.enum.ControlledReservoirEnergySpec2P.LiquidTemperature  area_A=0.1 m^2  pressure_limit_spec=foundation.enum.PressureLimitSpec2P.Limit
      settings: InternalSimscapePortConfiguration="{\"Bottom\":[],\"Left\":[{\"id\":\"A\",\"label\":\"A\",\"type\":\"foundation.two_phase_fluid.two_phase_fluid\"}],\"Right\":[{\"id\":\"T\",\"label\":\"T\",\"type\":\"input\"},{\"id\":\"P\",\"label\":\"P\",\"type\":\"input\"}],\"Top\":[]}"
  LH2 supply check valve : SimscapeFluids_lib/Two-Phase Fluid/Valves & Orifices/Directional Control Valves/Check Valve (2P)  liquid_valve_parameterization=fluids.two_phase_fluid.valves_orifices.enum.LiquidPressureValveParameterization.LinearArea  opening_pressure_spec=fluids.two_phase_fluid.valves_orifices.enum.PressureControlSpec.PressureDifferential  p_crack_differential=0.01 bar  p_crack_gauge=0.1 MPa  p_max_differential=0.03 bar  p_max_gauge=0.2 MPa  mdot_nominal_max=0.1 kg/s  delta_p_nominal_max=0.001 MPa  valve_area_max=supply_valve_orifice_area m^2  p_diff_TLU=[0.2 : 0.2 : 1.2] MPa  p_gauge_TLU=[0.2 : 0.2 : 1.2] MPa  valve_area_TLU=[1e-10, 2e-06, 4e-06, 6e-06, 8e-06, 1e-05] m^2  energy_spec=foundation.enum.energy_spec.temperature  p_inlet=0.101325 MPa  T_inlet=293.15 K  x_inlet=0  alpha_inlet=0  h_inlet=400 kJ/kg  u_inlet=400 kJ/kg  Cd=0.8  pressure_recovery=false  leakage_fraction=1e-9  smoothing_factor=0.01  B_lam=valve_laminar_p_ratio  tau_x=0.1 s  area=supply_pipe_inner_area m^2  vapor_valve_parameterization=fluids.two_phase_fluid.valves_orifices.enum.VaporOrificeParameterization.Cv  opening_characteristic=fluids.two_phase_fluid.valves_orifices.enum.OpeningCharacteristics.Linear  Cv_max=4  p_diff_Cv_TLU=0.2 : 0.2 : 1.2 MPa  p_gauge_Cv_TLU=0.2 : 0.2 : 1.2 MPa  Cv_TLU=[1e-06, .8, 1.6, 2.4, 3.2, 4]  xT_Cv=0.7  Kv_max=3.6  p_diff_Kv_TLU=0.2 : 0.2 : 1.2 MPa  p_gauge_Kv_TLU=0.2 : 0.2 : 1.2 MPa  Kv_TLU=[1e-06, .72, 1.44, 2.16, 2.88, 3.6]  xT_Kv=0.7  orifice_area_max=1e-4 m^2  p_diff_orifice_area_TLU=0.2 : 0.2 : 1.2 MPa  p_gauge_orifice_area_TLU=0.2 : 0.2 : 1.2 MPa  orifice_area_TLU=[1e-10, 2e-05, 4e-05, 6e-05, 8e-05, .0001] m^2
      settings: InternalSimscapePortConfiguration="{\"Bottom\":[],\"Left\":[{\"id\":\"A\",\"label\":\"A\",\"type\":\"foundation.two_phase_fluid.two_phase_fluid\"}],\"Right\":[{\"id\":\"B\",\"label\":\"B\",\"type\":\"foundation.two_phase_fluid.two_phase_fluid\"}],\"Top\":[]}"
  LH2 supply flow rate sensor : fl_lib/Two-Phase Fluid/Sensors/Flow Rate Sensor (2P)  mass_flow_measure=false  volumetric_flow_measure=true  energy_flow_measure=false
      settings: InternalSimscapePortConfiguration="{\"Bottom\":[],\"Left\":[{\"id\":\"A\",\"label\":\"A\",\"type\":\"foundation.two_phase_fluid.two_phase_fluid\"}],\"Right\":[{\"id\":\"B\",\"label\":\"B\",\"type\":\"foundation.two_phase_fluid.two_phase_fluid\"},{\"id\":\"V\",\"label\":\"V\",\"type\":\"output\"}],\"Top\":[]}"
  LH2 vent : fl_lib/Two-Phase Fluid/Sensors/Flow Rate Sensor (2P)  mass_flow_measure=false  volumetric_flow_measure=true  energy_flow_measure=false
      settings: InternalSimscapePortConfiguration="{\"Bottom\":[],\"Left\":[{\"id\":\"A\",\"label\":\"A\",\"type\":\"foundation.two_phase_fluid.two_phase_fluid\"}],\"Right\":[{\"id\":\"B\",\"label\":\"B\",\"type\":\"foundation.two_phase_fluid.two_phase_fluid\"},{\"id\":\"V\",\"label\":\"V\",\"type\":\"output\"}],\"Top\":[]}"
  LH2 vent proportional valve : Subsystem  ReferencedSubsystem=Return_gas_prop_valve
      settings: PortSchema="{\"entries\":[{\"content\":{\"sides\":[{\"content\":{\"connectorIds\":[\"LConn2\",\"In1\"]},\"type\":\"ConnectorPlacement.EquallySpacedRectSide\",\"uuid\":\"7b60590b-4a7b-465d-b616-9ce36d4c9bd1\"},{\"content\":{\"connectorIds\":[\"LConn1\",\"Out1\"],\"side\":\"RIGHT\"},\"type\":\"ConnectorPlacement.EquallySpacedRectSide\",\"uuid\":\"021f4d26-2a2b-40fc-b211-2c38ffe0620d\"},{\"content\":{\"side\":\"TOP\"},\"type\":\"ConnectorPlacement.EquallySpacedRectSide\",\"uuid\":\"273f71b8-2e8c-4f2f-b50f-0419d15b1792\"}]},\"type\":\"ConnectorPlacement.EquallySpacedConnector\",\"uuid\":\"b42a82ba-0baa-43b5-8ff8-ec1372f42070\"}],\"packageUris\":[\"http://schema.mathworks.com/mf0/Connector/R2020b\"],\"version\":\"1.0\"}"
  PS-Simulink Converter{,1,3..51} (51 alike) : nesl_utility/PS-Simulink Converter  PhysicalDomain=network_engine_domain  SubClassName=ps_output  LeftPortType=input  RightPortType=output  PseudoPeriodic=off  Frequencies=[]  VectorFormat=inherit  Unit=inherit  AffineConversion=off
  PS-Simulink Converter2 : nesl_utility/PS-Simulink Converter  Commented=on  PhysicalDomain=network_engine_domain  SubClassName=ps_output  LeftPortType=input  RightPortType=output  PseudoPeriodic=off  Frequencies=[]  VectorFormat=inherit  Unit=inherit  AffineConversion=off
  Pressure, Temperature & Internal Energy Sensor (2P){,1..13} (14 alike) : fl_lib/Two-Phase Fluid/Sensors/Pressure, Temperature & Internal Energy Sensor (2P)  reference=foundation.enum.MeasurementReference.absolute  pressure=true  pressure_spec=foundation.enum.PressureMeasementSpec.Absolute  temperature=true  internal_energy=false
      settings: InternalSimscapePortConfiguration="{\"Bottom\":[{\"id\":\"T\",\"label\":\"T\",\"type\":\"output\"}],\"Left\":[{\"id\":\"A\",\"label\":\"A\",\"type\":\"foundation.two_phase_fluid.two_phase_fluid\"}],\"Right\":[{\"id\":\"Pa\",\"label\":\"Pa\",\"type\":\"output\"}],\"Top\":[]}"
  Return line hose : Subsystem
  Safety valve : SimscapeFluids_lib/Two-Phase Fluid/Valves & Orifices/Directional Control Valves/Check Valve (2P)  Commented=on  liquid_valve_parameterization=fluids.two_phase_fluid.valves_orifices.enum.LiquidPressureValveParameterization.LinearArea  opening_pressure_spec=fluids.two_phase_fluid.valves_orifices.enum.PressureControlSpec.PressureDifferential  p_crack_differential=6 bar  p_crack_gauge=0.1 MPa  p_max_differential=7 bar  p_max_gauge=0.2 MPa  mdot_nominal_max=0.1 kg/s  delta_p_nominal_max=0.001 MPa  valve_area_max=1e-2 m^2  p_diff_TLU=[0.2 : 0.2 : 1.2] MPa  p_gauge_TLU=[0.2 : 0.2 : 1.2] MPa  valve_area_TLU=[1e-10, 2e-06, 4e-06, 6e-06, 8e-06, 1e-05] m^2  energy_spec=foundation.enum.energy_spec.temperature  p_inlet=0.101325 MPa  T_inlet=293.15 K  x_inlet=0  alpha_inlet=0  h_inlet=400 kJ/kg  u_inlet=400 kJ/kg  Cd=0.64  pressure_recovery=false  leakage_fraction=1e-9  smoothing_factor=0.01  B_lam=0.999  tau_x=0.1 s  area=0.02 m^2  vapor_valve_parameterization=fluids.two_phase_fluid.valves_orifices.enum.VaporOrificeParameterization.Cv  opening_characteristic=fluids.two_phase_fluid.valves_orifices.enum.OpeningCharacteristics.Linear  Cv_max=4  p_diff_Cv_TLU=0.2 : 0.2 : 1.2 MPa  p_gauge_Cv_TLU=0.2 : 0.2 : 1.2 MPa  Cv_TLU=[1e-06, .8, 1.6, 2.4, 3.2, 4]  xT_Cv=0.7  Kv_max=3.6  p_diff_Kv_TLU=0.2 : 0.2 : 1.2 MPa  p_gauge_Kv_TLU=0.2 : 0.2 : 1.2 MPa  Kv_TLU=[1e-06, .72, 1.44, 2.16, 2.88, 3.6]  xT_Kv=0.7  orifice_area_max=1e-4 m^2  p_diff_orifice_area_TLU=0.2 : 0.2 : 1.2 MPa  p_gauge_orifice_area_TLU=0.2 : 0.2 : 1.2 MPa  orifice_area_TLU=[1e-10, 2e-05, 4e-05, 6e-05, 8e-05, .0001] m^2
      settings: InternalSimscapePortConfiguration="{\"Bottom\":[],\"Left\":[{\"id\":\"A\",\"label\":\"A\",\"type\":\"foundation.two_phase_fluid.two_phase_fluid\"}],\"Right\":[{\"id\":\"B\",\"label\":\"B\",\"type\":\"foundation.two_phase_fluid.two_phase_fluid\"}],\"Top\":[]}"
  Safety vent valve{,1..6} (7 alike) : SimscapeFluids_lib/Two-Phase Fluid/Valves & Orifices/Directional Control Valves/Check Valve (2P)  liquid_valve_parameterization=fluids.two_phase_fluid.valves_orifices.enum.LiquidPressureValveParameterization.LinearArea  opening_pressure_spec=fluids.two_phase_fluid.valves_orifices.enum.PressureControlSpec.PressureDifferential  p_crack_differential=GS_vent_cracking_delta_P bar  p_crack_gauge=0.1 MPa  p_max_differential=GS_vent_open_delta_P bar  p_max_gauge=0.2 MPa  mdot_nominal_max=0.1 kg/s  delta_p_nominal_max=0.001 MPa  valve_area_max=GS_vent_orifice_area m^2  p_diff_TLU=[0.2 : 0.2 : 1.2] MPa  p_gauge_TLU=[0.2 : 0.2 : 1.2] MPa  valve_area_TLU=[1e-10, 2e-06, 4e-06, 6e-06, 8e-06, 1e-05] m^2  energy_spec=foundation.enum.energy_spec.temperature  p_inlet=0.101325 MPa  T_inlet=293.15 K  x_inlet=0  alpha_inlet=0  h_inlet=400 kJ/kg  u_inlet=400 kJ/kg  Cd=GS_vent_discharge_coeff  pressure_recovery=false  leakage_fraction=1e-9  smoothing_factor=0.01  B_lam=valve_laminar_p_ratio  tau_x=0.1 s  area=GS_vent_inner_area m^2  vapor_valve_parameterization=fluids.two_phase_fluid.valves_orifices.enum.VaporOrificeParameterization.Cv  opening_characteristic=fluids.two_phase_fluid.valves_orifices.enum.OpeningCharacteristics.Linear  Cv_max=4  p_diff_Cv_TLU=0.2 : 0.2 : 1.2 MPa  p_gauge_Cv_TLU=0.2 : 0.2 : 1.2 MPa  Cv_TLU=[1e-06, .8, 1.6, 2.4, 3.2, 4]  xT_Cv=0.7  Kv_max=3.6  p_diff_Kv_TLU=0.2 : 0.2 : 1.2 MPa  p_gauge_Kv_TLU=0.2 : 0.2 : 1.2 MPa  Kv_TLU=[1e-06, .72, 1.44, 2.16, 2.88, 3.6]  xT_Kv=0.7  orifice_area_max=1e-4 m^2  p_diff_orifice_area_TLU=0.2 : 0.2 : 1.2 MPa  p_gauge_orifice_area_TLU=0.2 : 0.2 : 1.2 MPa  orifice_area_TLU=[1e-10, 2e-05, 4e-05, 6e-05, 8e-05, .0001] m^2
      settings: InternalSimscapePortConfiguration="{\"Bottom\":[],\"Left\":[{\"id\":\"A\",\"label\":\"A\",\"type\":\"foundation.two_phase_fluid.two_phase_fluid\"}],\"Right\":[{\"id\":\"B\",\"label\":\"B\",\"type\":\"foundation.two_phase_fluid.two_phase_fluid\"}],\"Top\":[]}"
  Simulink-PS Converter{1..22} (22 alike) : nesl_utility/Simulink-PS Converter  PhysicalDomain=network_engine_domain  SubClassName=ps_input  LeftPortType=input  RightPortType=output  PseudoPeriodic=off  Frequencies=[]  NoiseDistribution=none  NoiseParameters=[]  Unit=1  AffineConversion=off  FilteringAndDerivatives=provide  SimscapeFilterOrder=1  InputFilterTimeConstant=0.001  UdotUserProvided=0
  Solver Configuration2 : nesl_utility/Solver Configuration  PhysicalDomain=network_engine_domain  SubClassName=solver  LeftPortType=input  RightPortType=generic  Tones=[]  Harmonics=[]  SimulateNoise=off  Profile=off  UseLocalSampling=off  EnableSwitchedLinearOptims=on  FrequencyDomain=off  UseCCode=off  RelTol=0.001  AbsTol=0.001  MinStep=1e-09  ToWorkspace=off  RevertToSquareIcSolve=off  NumHomotopyIterations=100  PhasorMode=off  PhasorModeNumHarmonics=1  ConsistencySolver=NEWTON_XTOL_AFTER_FTOL  IndexReductionMethod=DerivativeReplacement  DoDC=off  ResidualTolerance=1e-09  ConsistencyTolSource=GLOBAL  ConsistencyAbsTol=0.001  ConsistencyRelTol=0.001  ConsistencyTolFactor=1e-7  UseLocalSolver=off  LocalSolverChoice=NE_TRAPEZOIDAL_ADVANCER  ResolveIndetEquations=on  FunctionEvalNumThread=1  LocalSolverSampleTime=1e-3  DoFixedCost=off  MaxNonlinIter=3  MaxModeIter=2  ComputeImpulses=off  ImpulseIterations=2  LinearAlgebra=auto  LinearAlgebraNumThread=0  EquationFormulation=NE_TIME_EF  DelaysMemoryBudget=1024  AutomaticFiltering=on  FilteringTimeConstant=0.001  PartitionStorageMethod=AS_NEEDED  PartitionMemoryBudget=1024  PartitionMethod=ROBUST  MultibodyUseLocalSolver=off  MultibodyLocalSolverChoice=ODE1  MultibodyLocalSolverSampleTime=0.001
  Vent check valve : SimscapeFluids_lib/Two-Phase Fluid/Valves & Orifices/Directional Control Valves/Check Valve (2P)  liquid_valve_parameterization=fluids.two_phase_fluid.valves_orifices.enum.LiquidPressureValveParameterization.LinearArea  opening_pressure_spec=fluids.two_phase_fluid.valves_orifices.enum.PressureControlSpec.PressureDifferential  p_crack_differential=0.1 bar  p_crack_gauge=0.1 MPa  p_max_differential=0.3 bar  p_max_gauge=0.2 MPa  mdot_nominal_max=0.1 kg/s  delta_p_nominal_max=0.001 MPa  valve_area_max=return_valve_orifice_area m^2  p_diff_TLU=[0.2 : 0.2 : 1.2] MPa  p_gauge_TLU=[0.2 : 0.2 : 1.2] MPa  valve_area_TLU=[1e-10, 2e-06, 4e-06, 6e-06, 8e-06, 1e-05] m^2  energy_spec=foundation.enum.energy_spec.temperature  p_inlet=0.101325 MPa  T_inlet=293.15 K  x_inlet=0  alpha_inlet=0  h_inlet=400 kJ/kg  u_inlet=400 kJ/kg  Cd=GS_vent_discharge_coeff  pressure_recovery=false  leakage_fraction=1e-9  smoothing_factor=0.01  B_lam=valve_laminar_p_ratio  tau_x=0.1 s  area=return_pipe_inner_area m^2  vapor_valve_parameterization=fluids.two_phase_fluid.valves_orifices.enum.VaporOrificeParameterization.Cv  opening_characteristic=fluids.two_phase_fluid.valves_orifices.enum.OpeningCharacteristics.Linear  Cv_max=4  p_diff_Cv_TLU=0.2 : 0.2 : 1.2 MPa  p_gauge_Cv_TLU=0.2 : 0.2 : 1.2 MPa  Cv_TLU=[1e-06, .8, 1.6, 2.4, 3.2, 4]  xT_Cv=0.7  Kv_max=3.6  p_diff_Kv_TLU=0.2 : 0.2 : 1.2 MPa  p_gauge_Kv_TLU=0.2 : 0.2 : 1.2 MPa  Kv_TLU=[1e-06, .72, 1.44, 2.16, 2.88, 3.6]  xT_Kv=0.7  orifice_area_max=1e-4 m^2  p_diff_orifice_area_TLU=0.2 : 0.2 : 1.2 MPa  p_gauge_orifice_area_TLU=0.2 : 0.2 : 1.2 MPa  orifice_area_TLU=[1e-10, 2e-05, 4e-05, 6e-05, 8e-05, .0001] m^2
      settings: InternalSimscapePortConfiguration="{\"Bottom\":[],\"Left\":[{\"id\":\"A\",\"label\":\"A\",\"type\":\"foundation.two_phase_fluid.two_phase_fluid\"}],\"Right\":[{\"id\":\"B\",\"label\":\"B\",\"type\":\"foundation.two_phase_fluid.two_phase_fluid\"}],\"Top\":[]}"
  fuel cell : fl_lib/Two-Phase Fluid/Elements/Reservoir (2P)  pressure_spec=foundation.enum.ReservoirPressureSpec2P.Specified  reservoir_pressure=1.2 bar  reservoir_condensing_temperature=373.15 K  reservoir_evaporating_temperature=373.15 K  energy_spec=foundation.enum.ReservoirEnergySpec2P.Temperature  reservoir_temperature=Ambient_temp K  reservoir_quality=0.5  reservoir_void_fraction=0.5  reservoir_enthalpy=1500 kJ/kg  reservoir_internal_energy=1500 kJ/kg  reservoir_subcooling=5 deltaK  reservoir_superheating=5 deltaK  area_A=AC_engine_feed_port_inner_area m^2
  supply line hose : Subsystem
  mdot_ground_tank : Outport
  P_PUMP_GS : Outport  Port=2
  P_GH2_SUPPLY_GS : Outport  Port=3
  P_VALVE_RETURN_GS : Outport  Port=4
  T_BYPASS : Outport  Port=5
  Refuel_quality_check : Outport  Port=6
  AC_TK_LEVEL : Outport  Port=7
  P_TANK_AC : Outport  Port=8
  T_TANK_AC : Outport  Port=9
  P_BYPASS : Outport  Port=10
  P_COUPLING_AC : Outport  Port=11
  P_COUPLING_AC_RETURN : Outport  Port=12
  P_DIAGNOSTIC : Outport  Port=13  OutDataTypeStr=Bus: P_DIAGNOSTIC
  T_DIAGNOSTIC : Outport  Port=14  OutDataTypeStr=Bus: T_DIAGNOSTIC
  AC_TANK_SUPPLY_LINE_MDOT : Outport  Port=15
  LH2_SUPPLY_QDOT : Outport  Port=16
  GH2_SUPPLY_QDOT : Outport  Port=17
  GS_RETURN_QDOT : Outport  Port=18
  Engine_feed_mdot : Outport  Port=19
  AC_Tank_return_line_mdot : Outport  Port=20
  AC_Tank_Vent_mdot : Outport  Port=21
  Tank wall temp : Outport  Port=22
  GS_VALVE_FEEDBACK : Outport  Port=23  OutDataTypeStr=Bus: GS_VALVE_FEEDBACK
  AC_VALVE_FEEDBACK : Outport  Port=24  OutDataTypeStr=Bus: AC_VALVE_FEEDBACK
  AC_RETURN_VAPOUR_QUALITY : Outport  Port=25
  P_GAS_RETURN : Outport  Port=26
  P_HOSE_GS : Outport  Port=27
  P_HOSE_RETURN_GS : Outport  Port=28
  AC_QDOT : Outport  Port=29  OutDataTypeStr=Bus: AC_QDOT
  AC_MDOT : Outport  Port=30  OutDataTypeStr=Bus: AC_MDOT
  tag scope: P_GAS_RETURN=global
  wires:
  [GS_LH2_Return_SOV_CMD] -> GS LH2 Return SOV/1
  [AC_Bypass_SOV_CMD] -> AC_Bypass_SOV/1
  PS-Simulink Converter8/1 -> [P_TANK_GS]
  PS-Simulink Converter13/1 -> [T_HOSE_RETURN_GS]
  PS-Simulink Converter/1 -> [T_BYPASS]
  PS-Simulink Converter11/1 -> [Engine_feed_mdot]
  [AC_Engine_SOV_CMD] -> AC_Engine_SOV/1
  LH2 vent proportional valve/1 -> [GS_RETURN_PROP_POS]
  Constant1/1 -> Simulink-PS Converter3/1
  PS-Simulink Converter2/1 -> Goto1/1
  [Couplings_connected] -> AC_Return_Coupling/1
  PS-Simulink Converter23/1 -> [T_COUPLING_AC_RETURN]
  PS-Simulink Converter19/1 -> [P_COUPLINGS_GS]
  PS-Simulink Converter34/1 -> [P_ENGINE_FEED]
  PS-Simulink Converter25/1 -> [LH2_SUPPLY_QDOT]
  [Couplings_connected] -> AC_Supply_Coupling/1
  PS-Simulink Converter6/1 -> [P_TANK_AC]
  PS-Simulink Converter17/1 -> [P_HOSE_GS]
  GS_Supply_SOV/1 -> [GS_Supply_SOV_POS]
  PS-Simulink Converter10/1 -> [AC_TANK_SUPPLY_LINE_MDOT]
  PS-Simulink Converter37/1 -> [AC_Tank_Vent_mdot]
  PS-Simulink Converter20/1 -> [P_HOSE_RETURN_GS]
  Constant2/1 -> Simulink-PS Converter5/1
  PS-Simulink Converter7/1 -> [T_TANK_GS]
  [Couplings_connected] -> GS_Return_Coupling/1
  Constant5/1 -> Simulink-PS Converter2/1
  [LH2_PROP_VALVE_CMD] -> LH2 Proportional valve/1
  PS-Simulink Converter18/1 -> [T_COUPLINGS_GS]
  PS-Simulink Converter3/1 -> [AC_TK_LEVEL]
  [GS_LH2_Supply_SOV_CMD] -> GS_Supply_SOV/1
  AC_Return_SOV/1(VALVE_POS) -> [AC_Return_SOV_POS]
  PS-Simulink Converter15/1 -> [P_VALVE_GS]
  PS-Simulink Converter16/1 -> [T_HOSE_GS]
  AC tank/1 -> [TANK_WALL_TEMP]
  PS-Simulink Converter31/1 -> [P_PUMP_GS]
  PS-Simulink Converter30/1 -> [T_PUMP_GS]
  PS-Simulink Converter12/1 -> [T_VALVE_RETURN_GS]
  [LH2_VENT_PROP_VALVE_CMD] -> LH2 vent proportional valve/1
  LH2 Proportional valve/1 -> [LH2_PROP_VALVE_POS]
  PS-Simulink Converter21/1 -> [T_COUPLING_AC]
  PS-Simulink Converter22/1 -> [P_COUPLING_AC]
  PS-Simulink Converter4/1 -> [Refuel_quality_check]
  PS-Simulink Converter5/1 -> [T_TANK_AC]
  [AC_Supply_SOV_CMD] -> AC_Supply_SOV/1
  Constant4/1 -> Simulink-PS Converter4/1
  From/1 -> GS tank pressure controller/1(Target pressure)
  PS-Simulink Converter28/1 -> [GS_RETURN_QDOT]
  PS-Simulink Converter24/1 -> [P_COUPLING_AC_RETURN]
  PS-Simulink Converter14/1 -> [T_VALVE_GS]
  PS-Simulink Converter38/1 -> [AC_Tank_return_line_mdot]
  PS-Simulink Converter1/1 -> [mdot_ground_tank]
  GS LH2 Return SOV/1 -> [GS_LH2_Return_SOV_POS]
  AC_Supply_SOV/1 -> [AC_Supply_SOV_POS]
  PS-Simulink Converter27/1 -> [P_VALVE_RETURN_GS]
  [Couplings_connected] -> GS_Supply_Coupling/1
  PS-Simulink Converter33/1 -> [T_ENGINE_FEED]
  AC_Bypass_SOV/1 -> [AC_Bypass_SOV_POS]
  [AC_Return_SOV_CMD] -> AC_Return_SOV/1(Valve_command)
  AC_Engine_SOV/1 -> [AC_Engine_SOV_POS]
  PS-Simulink Converter9/1 -> [P_BYPASS]
  From14/1 -> GS tank pressure controller/2(Tank pressure)
  [GS_GH2_SOV_POS] -> Bus Assignment2/5
  AC_Bypass_SOV_CMD/1 -> [AC_Bypass_SOV_CMD]
  [AC_Tank_Vent_mdot] -> AC_Tank_Vent_mdot/1
  [T_BYPASS] -> T_BYPASS/1
  Couplings_connected/1 -> [Couplings_connected]
  [Engine_feed_mdot] -> Engine_feed_mdot/1
  [T_BYPASS] -> Bus Assignment1/9
  [AC_Bypass_SOV_POS] -> Bus Assignment3/4
  [P_VALVE_GS] -> Bus Assignment/5
  [P_TANK_AC] -> P_TANK_AC/1
  [P_VALVE_RETURN_GS] -> P_VALVE_RETURN_GS/1
  [T_ENGINE_FEED] -> Bus Assignment1/11
  AC_Engine_SOV_CMD/1 -> [AC_Engine_SOV_CMD]
  [P_HOSE_RETURN_GS] -> Bus Assignment/13
  GS_GH2_SOV_CMD/1 -> [GS_GH2_SOV_CMD]
  GH2_PROP_VALVE_CMD/1 -> [GH2_PROP_VALVE_CMD]
  [P_COUPLING_AC_RETURN] -> Bus Assignment/12
  AC_Supply_SOV_CMD/1 -> [AC_Supply_SOV_CMD]
  [P_TANK_AC] -> Bus Assignment/10
  LH2_PROP_VALVE_CMD/1 -> [LH2_PROP_VALVE_CMD]
  [GH2_PROP_VALVE_POS] -> Bus Assignment2/3
  Bus Assignment1/1 -> T_DIAGNOSTIC/1
  [GS_LH2_Return_SOV_POS] -> Bus Assignment2/6
  [TANK_WALL_TEMP] -> Tank wall temp/1
  [T_COUPLING_AC] -> Bus Assignment1/8
  [T_COUPLINGS_GS] -> Bus Assignment1/7
  [T_PUMP_GS] -> Bus Assignment1/3
  [T_GH2_SUPPLY_GS] -> Bus Assignment1/4
  [Refuel_quality_check] -> Refuel_quality_check/1
  [T_TANK_GS] -> Bus Assignment1/2
  [P_COUPLING_AC_RETURN] -> P_COUPLING_AC_RETURN/1
  [P_BYPASS] -> Bus Assignment/9
  [GS_RETURN_QDOT] -> GS_RETURN_QDOT/1
  [T_COUPLING_AC_RETURN] -> Bus Assignment1/12
  [P_ENGINE_FEED] -> Bus Assignment/11
  [P_COUPLING_AC] -> P_COUPLING_AC/1
  GS_LH2_Supply_SOV_CMD/1 -> [GS_LH2_Supply_SOV_CMD]
  [T_VALVE_RETURN_GS] -> Bus Assignment1/14
  [mdot_ground_tank] -> mdot_ground_tank/1
  Bus Creator/1 -> Bus Assignment/1
  Bus Assignment2/1 -> GS_VALVE_FEEDBACK/1
  [P_COUPLING_AC] -> Bus Assignment/8
  [LH2_PROP_VALVE_POS] -> Bus Assignment2/2
  [P_PUMP_GS] -> Bus Assignment/3
  [P_GH2_SUPPLY_GS] -> Bus Assignment/4
  [AC_Return_SOV_POS] -> Bus Assignment3/2
  [P_TANK_GS] -> Bus Assignment/2
  [P_BYPASS] -> P_BYPASS/1
  [AC_Engine_SOV_POS] -> Bus Assignment3/5
  [AC_TK_LEVEL] -> AC_TK_LEVEL/1
  LH2 VENT PROP VALVE CMD/1 -> [LH2_VENT_PROP_VALVE_CMD]
  Bus Assignment/1 -> P_DIAGNOSTIC/1
  AC_Return_SOV_CMD/1 -> [AC_Return_SOV_CMD]
  [P_PUMP_GS] -> P_PUMP_GS/1
  [T_VALVE_GS] -> Bus Assignment1/5
  [T_HOSE_RETURN_GS] -> Bus Assignment1/13
  [GS_Supply_SOV_POS] -> Bus Assignment2/4
  [P_COUPLINGS_GS] -> Bus Assignment/7
  [AC_TANK_SUPPLY_LINE_MDOT] -> AC_TANK_SUPPLY_LINE_MDOT/1
  Bus Assignment3/1 -> AC_VALVE_FEEDBACK/1
  [AC_Supply_SOV_POS] -> Bus Assignment3/3
  Bus Creator2/1 -> Bus Assignment2/1
  [AC_Tank_return_line_mdot] -> AC_Tank_return_line_mdot/1
  [GS_RETURN_PROP_POS] -> Bus Assignment2/7
  [T_TANK_AC] -> T_TANK_AC/1
  [T_HOSE_GS] -> Bus Assignment1/6
  GS_LH2_Return_SOV_CMD/1 -> [GS_LH2_Return_SOV_CMD]
  Bus Creator3/1 -> Bus Assignment3/1
  [P_HOSE_GS] -> Bus Assignment/6
  [GH2_SUPPLY_QDOT] -> GH2_SUPPLY_QDOT/1
  [T_TANK_AC] -> Bus Assignment1/10
  [P_VALVE_RETURN_GS] -> Bus Assignment/14
  Bus Creator1/1 -> Bus Assignment1/1
  [LH2_SUPPLY_QDOT] -> LH2_SUPPLY_QDOT/1
  [P_GH2_SUPPLY_GS] -> P_GH2_SUPPLY_GS/1
  Constant3/1 -> Simulink-PS Converter7/1
  Constant7/1 -> Simulink-PS Converter6/1
  PS-Simulink Converter29/1 -> [AC_RETURN_VAPOUR_QUALITY]
  [AC_RETURN_VAPOUR_QUALITY] -> AC_RETURN_VAPOUR_QUALITY/1
  Constant8/1 -> Simulink-PS Converter9/1
  [GS_GH2_SOV_CMD] -> GS GH2 SOV/1
  PS-Simulink Converter39/1 -> [T_GH2_SUPPLY_GS]
  GS GH2 SOV/1 -> [GS_GH2_SOV_POS]
  GH2 Proportional valve/1 -> [GH2_PROP_VALVE_POS]
  PS-Simulink Converter40/1 -> [P_GH2_SUPPLY_GS]
  Constant9/1 -> Simulink-PS Converter8/1
  [GH2_PROP_VALVE_CMD] -> GH2 Proportional valve/1
  PS-Simulink Converter32/1 -> [GH2_SUPPLY_QDOT]
  Constant6/1 -> Simulink-PS Converter10/1
  Constant10/1 -> Simulink-PS Converter1/1
  PS-Simulink Converter26/1 -> [T_GAS_RETURN]
  PS-Simulink Converter35/1 -> [P_GAS_RETURN]
  [GS_GH2_RETURN_SOV_CMD] -> GS_GH2_Return/1
  [GH2_VENT_PROP_VALVE_CMD] -> GH2 vent proportional valve/1
  [P_GAS_RETURN] -> Bus Assignment/15
  [T_GAS_RETURN] -> Bus Assignment1/15
  GH2 vent proportional valve/1 -> [GS_GH2_RETURN_PROP_POS]
  GS_GH2_Return/1 -> [GS_GH2_RETURN_SOV_POS]
  [GS_GH2_RETURN_PROP_POS] -> Bus Assignment2/8
  [GS_GH2_RETURN_SOV_POS] -> Bus Assignment2/9
  GS_GH2_RETURN_SOV_CMD/1 -> [GS_GH2_RETURN_SOV_CMD]
  GH2_VENT_PROP_VALVE_CMD/1 -> [GH2_VENT_PROP_VALVE_CMD]
  [P_GAS_RETURN] -> P_GAS_RETURN/1
  [P_HOSE_GS] -> P_HOSE_GS/1
  [P_HOSE_RETURN_GS] -> P_HOSE_RETURN_GS/1
  PS-Simulink Converter36/1 -> [AC_TANK_SUPPLY_LINE_QDOT]
  PS-Simulink Converter41/1 -> [Engine_feed_Qdot]
  PS-Simulink Converter42/1 -> [AC_Tank_Vent_Qdot]
  PS-Simulink Converter43/1 -> [AC_Tank_return_line_Qdot]
  PS-Simulink Converter44/1 -> [AC_return_coupling_Qdot]
  PS-Simulink Converter45/1 -> [AC_supply_coupling_Qdot]
  PS-Simulink Converter46/1 -> [AC_bypass_line_Qdot]
  Bus Creator4/1 -> Bus Assignment4/1
  [AC_bypass_line_Qdot] -> Bus Assignment4/6
  [AC_supply_coupling_Qdot] -> Bus Assignment4/5
  [AC_return_coupling_Qdot] -> Bus Assignment4/4
  [AC_Tank_return_line_Qdot] -> Bus Assignment4/7
  [AC_TANK_SUPPLY_LINE_QDOT] -> Bus Assignment4/8
  [Engine_feed_Qdot] -> Bus Assignment4/9
  [AC_Tank_Vent_Qdot] -> Bus Assignment4/10
  Bus Assignment4/1 -> AC_QDOT/1
  PS-Simulink Converter47/1 -> [AC_supply_line_Qdot]
  [AC_supply_line_Qdot] -> Bus Assignment4/2
  [AC_return_line_Qdot] -> Bus Assignment4/3
  PS-Simulink Converter48/1 -> [AC_return_line_Qdot]
  PS-Simulink Converter49/1 -> [AC_supply_line_Mdot]
  PS-Simulink Converter50/1 -> [AC_bypass_line_Mdot]
  PS-Simulink Converter51/1 -> [AC_return_line_Mdot]
  Bus Creator5/1 -> Bus Assignment5/1
  Bus Assignment5/1 -> AC_MDOT/1
  [AC_supply_line_Mdot] -> Bus Assignment5/2
  [AC_bypass_line_Mdot] -> Bus Assignment5/3
  [AC_return_line_Mdot] -> Bus Assignment5/4
  [AC_Tank_return_line_mdot] -> Bus Assignment5/5
  [AC_Tank_Vent_mdot] -> Bus Assignment5/7
  [Engine_feed_mdot] -> Bus Assignment5/8
  [AC_TANK_SUPPLY_LINE_MDOT] -> Bus Assignment5/6
  Constant14/1 -> Simulink-PS Converter13/1
  Constant13/1 -> Simulink-PS Converter14/1
  Constant12/1 -> Simulink-PS Converter11/1
  Constant11/1 -> Simulink-PS Converter12/1
  Constant16/1 -> Simulink-PS Converter15/1
  Constant15/1 -> Simulink-PS Converter16/1
  Constant18/1 -> Simulink-PS Converter17/1
  Constant17/1 -> Simulink-PS Converter18/1
  Constant19/1 -> Simulink-PS Converter20/1
  Constant20/1 -> Simulink-PS Converter19/1
  Constant21/1 -> Simulink-PS Converter22/1
  Constant22/1 -> Simulink-PS Converter21/1
  connections:
  "Pressure, Temperature & Internal Energy Sensor (2P)2"/LConn1 -- Solver Configuration2/RConn1 -- H2 2 phase/RConn1 -- Ground station tank/LConn2 -- LH2 source/LConn1 -- Ground station tank/RConn2 -- LH2 Proportional valve/LConn1
  AC bypass pipe/RConn1 -- AC return vapour quality/LConn1 -- Flow Rate Sensor (2P)4/LConn1 -- AC_Return_SOV/LConn1
  "Pressure, Temperature & Internal Energy Sensor (2P)7"/LConn1 -- AC_Supply_Coupling/LConn1 -- GS_Supply_Coupling/RConn1
  Safety vent valve6/LConn1 -- GS LH2 Return SOV/RConn1 -- Return line hose/LConn1 -- GH2 supply check valve/RConn1
  AC engine feed pipe/LConn1 -- "Pressure, Temperature & Internal Energy Sensor (2P)11"/LConn1 -- Flow Rate Sensor (2P)3/RConn1
  Flow Rate Sensor (2P)8/LConn1 -- AC return line pipe/LConn1 -- "Pressure, Temperature & Internal Energy Sensor (2P)9"/LConn1
  "Pressure, Temperature & Internal Energy Sensor (2P)6"/LConn1 -- GS_Supply_Coupling/LConn1 -- supply line hose/RConn1
  AC supply line quality/LConn1 -- Flow Rate Sensor (2P)2/LConn1 -- AC_Supply_SOV/RConn1 -- "Pressure, Temperature & Internal Energy Sensor (2P)1"/LConn1
  Flow Rate Sensor (2P)10/LConn1 -- AC_Supply_SOV/LConn1 -- Flow Rate Sensor (2P)1/RConn1 -- "Pressure, Temperature & Internal Energy Sensor (2P)"/LConn1
  "Pressure, Temperature & Internal Energy Sensor (2P)10"/LConn1 -- Safety vent valve2/LConn1 -- GS_Supply_SOV/LConn1 -- GS supply line pipe/RConn1
  GS return line pipe short/RConn1 -- "Pressure, Temperature & Internal Energy Sensor (2P)13"/LConn1 -- GS GH2 SOV/LConn1
  "Pressure, Temperature & Internal Energy Sensor (2P)12"/LConn1 -- GS_GH2_Return/LConn1 -- Safety vent valve4/LConn1 -- GS supply line pipe1/RConn1
  Safety vent valve3/LConn1 -- GH2 return check valve/LConn1 -- supply line hose/LConn1 -- LH2 supply check valve/RConn1 -- Safety vent valve/LConn1
  GS supply line pipe short1/LConn1 -- LH2 supply flow rate sensor/RConn1 -- Safety vent valve1/LConn1 -- "Pressure, Temperature & Internal Energy Sensor (2P)5"/LConn1
  "Pressure, Temperature & Internal Energy Sensor (2P)3"/LConn1 -- GS return line pipe short2/RConn1 -- GS LH2 Return SOV/LConn1
  "Pressure, Temperature & Internal Energy Sensor (2P)4"/LConn1 -- GS_Return_Coupling/LConn1 -- Return line hose/RConn1
  "Pressure, Temperature & Internal Energy Sensor (2P)8"/LConn1 -- AC_supply_line_pipe/LConn1 -- Flow Rate Sensor (2P)9/RConn1
  GS return line pipe short2/LConn1 -- Safety vent valve5/LConn1 -- LH2 vent proportional valve/LConn1
  Safety vent valve2/RConn1 -- GH2 vent1/LConn1
  GH2 vent/LConn1 -- Vent check valve/RConn1
  GH2 return check valve/RConn1 -- GS_GH2_Return/RConn1
  Flow Rate Sensor (2P)9/LConn1 -- AC_Supply_Coupling/RConn1
  LH2 supply check valve/LConn1 -- GS supply line pipe short1/RConn1
  GH2 vent proportional valve/LConn1 -- GS supply line pipe1/LConn1
  PS-Simulink Converter17/LConn1 -- "Pressure, Temperature & Internal Energy Sensor (2P)6"/RConn1
  PS-Simulink Converter33/LConn1 -- "Pressure, Temperature & Internal Energy Sensor (2P)11"/RConn2
  AC_Engine_SOV/RConn1 -- Flow Rate Sensor (2P)3/LConn1
  PS-Simulink Converter3/LConn1 -- AC tank/RConn3
  AC tank safety valve/RConn1 -- Atmosphere2/LConn1
  AC_Return_Coupling/LConn1 -- GS_Return_Coupling/RConn1
  PS-Simulink Converter27/LConn1 -- "Pressure, Temperature & Internal Energy Sensor (2P)3"/RConn1
  PS-Simulink Converter4/LConn1 -- AC supply line quality/RConn1
  GH2 vent/RConn2 -- Simulink-PS Converter2/RConn1
  AC bypass pipe/LConn1 -- AC_Bypass_SOV/RConn1
  PS-Simulink Converter8/LConn1 -- "Pressure, Temperature & Internal Energy Sensor (2P)2"/RConn1
  LH2 vent/LConn1 -- LH2 vent proportional valve/LConn2
  PS-Simulink Converter2/LConn1 -- Ground station tank/RConn3
  PS-Simulink Converter34/LConn1 -- "Pressure, Temperature & Internal Energy Sensor (2P)11"/RConn1
  PS-Simulink Converter14/LConn1 -- "Pressure, Temperature & Internal Energy Sensor (2P)5"/RConn2
  AC_Return_SOV/RConn1 -- Flow Rate Sensor (2P)6/RConn1
  AC_Engine_SOV/LConn1 -- AC tank/RConn2
  Safety valve/LConn1 -- Ground station tank/LConn1
  PS-Simulink Converter28/LConn1 -- LH2 vent/RConn2
  PS-Simulink Converter/LConn1 -- "Pressure, Temperature & Internal Energy Sensor (2P)"/RConn2
  PS-Simulink Converter19/LConn1 -- "Pressure, Temperature & Internal Energy Sensor (2P)7"/RConn1
  PS-Simulink Converter6/LConn1 -- "Pressure, Temperature & Internal Energy Sensor (2P)1"/RConn1
  AC engine feed pipe/RConn1 -- fuel cell/LConn1
  PS-Simulink Converter9/LConn1 -- "Pressure, Temperature & Internal Energy Sensor (2P)"/RConn1
  PS-Simulink Converter1/LConn1 -- Flow rate sensor/RConn2
  PS-Simulink Converter13/LConn1 -- "Pressure, Temperature & Internal Energy Sensor (2P)4"/RConn2
  PS-Simulink Converter38/LConn1 -- Flow Rate Sensor (2P)6/RConn2
  PS-Simulink Converter31/LConn1 -- "Pressure, Temperature & Internal Energy Sensor (2P)10"/RConn1
  PS-Simulink Converter21/LConn1 -- "Pressure, Temperature & Internal Energy Sensor (2P)8"/RConn2
  PS-Simulink Converter25/LConn1 -- LH2 supply flow rate sensor/RConn2
  PS-Simulink Converter11/LConn1 -- Flow Rate Sensor (2P)3/RConn2
  Vent check valve/LConn1 -- LH2 vent/RConn1
  PS-Simulink Converter24/LConn1 -- "Pressure, Temperature & Internal Energy Sensor (2P)9"/RConn1
  PS-Simulink Converter18/LConn1 -- "Pressure, Temperature & Internal Energy Sensor (2P)7"/RConn2
  PS-Simulink Converter7/LConn1 -- "Pressure, Temperature & Internal Energy Sensor (2P)2"/RConn2
  PS-Simulink Converter15/LConn1 -- "Pressure, Temperature & Internal Energy Sensor (2P)5"/RConn1
  PS-Simulink Converter20/LConn1 -- "Pressure, Temperature & Internal Energy Sensor (2P)4"/RConn1
  AC tank/RConn1 -- Flow Rate Sensor (2P)5/LConn1
  LH2 source/RConn2 -- Simulink-PS Converter4/RConn1
  PS-Simulink Converter22/LConn1 -- "Pressure, Temperature & Internal Energy Sensor (2P)8"/RConn1
  Flow Rate Sensor (2P)5/RConn1 -- AC tank safety valve/LConn1
  PS-Simulink Converter16/LConn1 -- "Pressure, Temperature & Internal Energy Sensor (2P)6"/RConn2
  Flow Rate Sensor (2P)2/RConn1 -- AC tank/LConn2
  Safety valve/RConn1 -- Atmosphere/LConn1
  PS-Simulink Converter5/LConn1 -- "Pressure, Temperature & Internal Energy Sensor (2P)1"/RConn2
  Simulink-PS Converter3/RConn1 -- LH2 source/RConn1
  Flow Rate Sensor (2P)6/LConn1 -- AC tank/LConn1
  PS-Simulink Converter37/LConn1 -- Flow Rate Sensor (2P)5/RConn2
  Simulink-PS Converter5/RConn1 -- GH2 vent/RConn1
  PS-Simulink Converter23/LConn1 -- "Pressure, Temperature & Internal Energy Sensor (2P)9"/RConn2
  PS-Simulink Converter12/LConn1 -- "Pressure, Temperature & Internal Energy Sensor (2P)3"/RConn2
  PS-Simulink Converter10/LConn1 -- Flow Rate Sensor (2P)2/RConn2
  PS-Simulink Converter30/LConn1 -- "Pressure, Temperature & Internal Energy Sensor (2P)10"/RConn2
  GS supply line pipe/LConn1 -- LH2 Proportional valve/LConn2
  GH2 vent1/RConn2 -- Simulink-PS Converter6/RConn1
  Simulink-PS Converter7/RConn1 -- GH2 vent1/RConn1
  PS-Simulink Converter29/LConn1 -- AC return vapour quality/RConn1
  GH2 Proportional valve/LConn1 -- GH2 source1/LConn1
  GS GH2 SOV/RConn1 -- Flow Rate Sensor (2P)7/LConn1
  PS-Simulink Converter40/LConn1 -- "Pressure, Temperature & Internal Energy Sensor (2P)13"/RConn1
  Flow Rate Sensor (2P)7/RConn2 -- PS-Simulink Converter32/LConn1
  Simulink-PS Converter8/RConn1 -- GH2 source1/RConn2
  Simulink-PS Converter9/RConn1 -- GH2 source1/RConn1
  PS-Simulink Converter39/LConn1 -- "Pressure, Temperature & Internal Energy Sensor (2P)13"/RConn2
  LH2 recycle/RConn2 -- Simulink-PS Converter1/RConn1
  Simulink-PS Converter10/RConn1 -- LH2 recycle/RConn1
  LH2 recycle/LConn1 -- GH2 return check valve1/RConn1
  PS-Simulink Converter35/LConn1 -- "Pressure, Temperature & Internal Energy Sensor (2P)12"/RConn1
  PS-Simulink Converter26/LConn1 -- "Pressure, Temperature & Internal Energy Sensor (2P)12"/RConn2
  GS return line pipe short/LConn1 -- GH2 Proportional valve/LConn2
  Flow Rate Sensor (2P)7/RConn1 -- GH2 supply check valve/LConn1
  Flow Rate Sensor (2P)2/RConn3 -- PS-Simulink Converter36/LConn1
  PS-Simulink Converter41/LConn1 -- Flow Rate Sensor (2P)3/RConn3
  PS-Simulink Converter42/LConn1 -- Flow Rate Sensor (2P)5/RConn3
  PS-Simulink Converter43/LConn1 -- Flow Rate Sensor (2P)6/RConn3
  Flow Rate Sensor (2P)8/RConn1 -- AC_Return_Coupling/RConn1
  Flow Rate Sensor (2P)8/RConn3 -- PS-Simulink Converter44/LConn1
  PS-Simulink Converter45/LConn1 -- Flow Rate Sensor (2P)9/RConn3
  AC_Bypass_SOV/LConn1 -- Flow Rate Sensor (2P)10/RConn1
  PS-Simulink Converter46/LConn1 -- Flow Rate Sensor (2P)10/RConn3
  GH2 return check valve1/LConn1 -- GH2 vent proportional valve/LConn2
  Flow rate sensor/RConn1 -- LH2 supply flow rate sensor/LConn1
  Flow rate sensor/LConn1 -- GS_Supply_SOV/RConn1
  Flow Rate Sensor (2P)1/LConn1 -- AC_supply_line_pipe/RConn1
  Flow Rate Sensor (2P)4/RConn1 -- AC return line pipe/RConn1
  PS-Simulink Converter48/LConn1 -- Flow Rate Sensor (2P)4/RConn3
  Flow Rate Sensor (2P)1/RConn3 -- PS-Simulink Converter47/LConn1
  PS-Simulink Converter49/LConn1 -- Flow Rate Sensor (2P)1/RConn2
  Flow Rate Sensor (2P)10/RConn2 -- PS-Simulink Converter50/LConn1
  Flow Rate Sensor (2P)4/RConn2 -- PS-Simulink Converter51/LConn1
  Safety vent valve4/RConn1 -- GH2 vent3/LConn1
  GH2 vent3/RConn2 -- Simulink-PS Converter13/RConn1
  Simulink-PS Converter14/RConn1 -- GH2 vent3/RConn1
  Safety vent valve5/RConn1 -- GH2 vent2/LConn1
  GH2 vent2/RConn2 -- Simulink-PS Converter11/RConn1
  Simulink-PS Converter12/RConn1 -- GH2 vent2/RConn1
  GH2 vent4/RConn2 -- Simulink-PS Converter15/RConn1
  Simulink-PS Converter16/RConn1 -- GH2 vent4/RConn1
  Safety vent valve/RConn1 -- GH2 vent4/LConn1
  GH2 vent5/RConn2 -- Simulink-PS Converter17/RConn1
  Simulink-PS Converter18/RConn1 -- GH2 vent5/RConn1
  GH2 vent5/LConn1 -- Safety vent valve1/RConn1
  GH2 vent6/RConn2 -- Simulink-PS Converter19/RConn1
  Simulink-PS Converter20/RConn1 -- GH2 vent6/RConn1
  Safety vent valve3/RConn1 -- GH2 vent6/LConn1
  Simulink-PS Converter22/RConn1 -- GH2 vent7/RConn1
  GH2 vent7/RConn2 -- Simulink-PS Converter21/RConn1
  GH2 vent7/LConn1 -- Safety vent valve6/RConn1
